simulink model "Test2_2"  (R2021a)
(part 2 of 3)

  Line 178 : spsDistributedParametersLineLib/Distributed Parameters Line  Phases=3  Length=0.02  Frequency=50  Resistance=[0.646656091154803 0.0486237908083191 0.0486712220507153;0.0486237908083191 0.646561225344642 0.0486237934466192;0.0486712220507153 0.0486237934466192 0.646656091154803]  Inductance=[0.00282448912315926 0.00133270803418135 0.00132951476746136;0.00133270803418135 0.00282479813276775 0.00133799988507366;0.00132951476746136 0.00133799988507366 0.00282448912315926]  Capacitance=[7.89543174552926e-09 -1.85986777702161e-09 -1.7901190036642e-09;-1.85986777702161e-09 7.82540023894543e-09 -1.8957321828871e-09;-1.7901190036642e-09 -1.8957321828871e-09 7.91264394645417e-09]  x1=[132.760320780997 9780.39904958768 9780.48623798031;314.159265358979 314.159265358979 314.159265358979;1.01437748390424 -0.192488813536579 -1.76345330045066]  x2=[132.762640557686 9780.24311209195 9780.33092876166;314.159265358979 314.159265358979 314.159265358979;1.01437617109871 -0.192497610718672 -1.7634621098678]  x3=[0.148387535223296 13.4653889012838 13.6374305581098;314.159265358979 314.159265358979 314.159265358979;0.608049237389297 -0.0518272275363164 -1.62927252881615]  x4=[0.112365930559543 36.4950552140708 36.6918967608298;314.159265358979 314.159265358979 314.159265358979;1.56346628767465 -0.244262443878478 -1.81321823531052]  x5=9.5829454252223e-08  V1=ones(3,3)  V2=ones(3,3)  I1=ones(3,3)  I2=ones(3,3)  nHarmo=1  Measurements=None  Decoupling=off  VsMag0=0  VrMag0=0  VsAngle0=0  VrAngle0=0  IsMag0=0  IrMag0=0  IsAngle0=0  IrAngle0=0
      settings: SourceProductBaseCode=PS
  Line 179 : spsDistributedParametersLineLib/Distributed Parameters Line  Phases=3  Length=1.15  Frequency=50  Resistance=[0.646656091154803 0.0486237908083191 0.0486712220507153;0.0486237908083191 0.646561225344642 0.0486237934466192;0.0486712220507153 0.0486237934466192 0.646656091154803]  Inductance=[0.00282448912315926 0.00133270803418135 0.00132951476746136;0.00133270803418135 0.00282479813276775 0.00133799988507366;0.00132951476746136 0.00133799988507366 0.00282448912315926]  Capacitance=[7.89543174552926e-09 -1.85986777702161e-09 -1.7901190036642e-09;-1.85986777702161e-09 7.82540023894543e-09 -1.8957321828871e-09;-1.7901190036642e-09 -1.8957321828871e-09 7.91264394645417e-09]  x1=[132.760320780997 9780.39904958768 9780.4862379803;314.159265358979 314.159265358979 314.159265358979;1.0126765112357 -0.193840124605235 -1.76480589787176]  x2=[132.768895455589 9779.25512812822 9779.34440600344;314.159265358979 314.159265358979 314.159265358979;1.01270315248622 -0.193874930127169 -1.76484031870729]  x3=[0.119132447239703 23.5945130394912 23.7849338463872;314.159265358979 314.159265358979 314.159265358979;0.986640133034939 -0.173292086707206 -1.74446117743403]  x4=[0.112976783804386 26.1275376195522 26.3187826598894;314.159265358979 314.159265358979 314.159265358979;1.03838062207725 -0.213738048990041 -1.78453527997739]  x5=5.51019361950282e-06  V1=ones(3,3)  V2=ones(3,3)  I1=ones(3,3)  I2=ones(3,3)  nHarmo=1  Measurements=None  Decoupling=off  VsMag0=0  VrMag0=0  VsAngle0=0  VrAngle0=0  IsMag0=0  IrMag0=0  IsAngle0=0  IrAngle0=0
      settings: SourceProductBaseCode=PS
  Line 18 : spsDistributedParametersLineLib/Distributed Parameters Line  Phases=3  Length=0.23002  Frequency=50  Resistance=[0.476003738225748 0.351747138225748 0.351747138225748;0.351747138225748 0.476003738225748 0.351747138225748;0.351747138225748 0.351747138225748 0.476003738225748]  Inductance=[0.000705954362986426 0.000459934243504405 0.000459934243504405;0.000459934243504405 0.000705954362986426 0.000459934243504405;0.000459934243504405 0.000459934243504405 0.000705954362986426]  Capacitance=[5.7561313269996e-07 -1.37543883484145e-07 -1.37543912800485e-07;-1.37543883484145e-07 5.75613027339387e-07 -1.37543875208088e-07;-1.37543912800485e-07 -1.37543875208088e-07 5.75613005057695e-07]  x1=[3.71917240590445 9847.49146197163 9847.74083952394;314.159265358979 314.159265358979 314.159265358979;1.3084049652874 2.1767138521056 -2.53557965242628]  x2=[3.71917715052359 9847.49597307011 9847.74535073597;314.159265358979 314.159265358979 314.159265358979;1.30840201930712 2.1767131156343 -2.53558038889746]  x3=[0.0504254137239255 529.580365853532 529.593736036669;314.159265358979 314.159265358979 314.159265358979;1.30680616940855 2.17575630443441 -2.53653720002242]  x4=[0.0504254137677653 529.58036594773 529.593736129492;314.159265358979 314.159265358979 314.159265358979;1.30840201941079 2.17671311563465 -2.53558038889797]  x5=5.08443513939426e-06  V1=ones(3,3)  V2=ones(3,3)  I1=ones(3,3)  I2=ones(3,3)  nHarmo=1  Measurements=None  Decoupling=off  VsMag0=0  VrMag0=0  VsAngle0=0  VrAngle0=0  IsMag0=0  IrMag0=0  IsAngle0=0  IrAngle0=0
      settings: SourceProductBaseCode=PS
  Line 180 : spsDistributedParametersLineLib/Distributed Parameters Line  Phases=3  Length=0.19  Frequency=50  Resistance=[0.646656091154803 0.0486237908083191 0.0486712220507153;0.0486237908083191 0.646561225344642 0.0486237934466192;0.0486712220507153 0.0486237934466192 0.646656091154803]  Inductance=[0.00282448912315926 0.00133270803418135 0.00132951476746136;0.00133270803418135 0.00282479813276775 0.00133799988507366;0.00132951476746136 0.00133799988507366 0.00282448912315926]  Capacitance=[7.89543174552926e-09 -1.85986777702161e-09 -1.7901190036642e-09;-1.85986777702161e-09 7.82540023894543e-09 -1.8957321828871e-09;-1.7901190036642e-09 -1.8957321828871e-09 7.91264394645417e-09]  x1=[132.768895455589 9779.25512812822 9779.34440600344;314.159265358979 314.159265358979 314.159265358979;1.01414822661171 -0.192726913644063 -1.76369120939378]  x2=[132.769311497012 9779.19565973239 9779.28506308661;314.159265358979 314.159265358979 314.159265358979;1.01414926755144 -0.192727707419426 -1.76369198402374]  x3=[0.116896171265332 24.525871144399 24.717022211576;314.159265358979 314.159265358979 314.159265358979;1.00614674760907 -0.184195073380317 -1.75522965039059]  x4=[0.115258964799221 25.2392564131172 25.4306773509319;314.159265358979 314.159265358979 314.159265358979;1.0219763695912 -0.201242395673975 -1.77214032483868]  x5=9.10379815396118e-07  V1=ones(3,3)  V2=ones(3,3)  I1=ones(3,3)  I2=ones(3,3)  nHarmo=1  Measurements=None  Decoupling=off  VsMag0=0  VrMag0=0  VsAngle0=0  VrAngle0=0  IsMag0=0  IrMag0=0  IsAngle0=0  IrAngle0=0
      settings: SourceProductBaseCode=PS
  Line 181 : spsDistributedParametersLineLib/Distributed Parameters Line  Phases=3  Length=0.34002  Frequency=50  Resistance=[0.646656091154803 0.0486237908083191 0.0486712220507153;0.0486237908083191 0.646561225344642 0.0486237934466192;0.0486712220507153 0.0486237934466192 0.646656091154803]  Inductance=[0.00282448912315926 0.00133270803418135 0.00132951476746136;0.00133270803418135 0.00282479813276775 0.00133799988507366;0.00132951476746136 0.00133799988507366 0.00282448912315926]  Capacitance=[7.89543174552926e-09 -1.85986777702161e-09 -1.7901190036642e-09;-1.85986777702161e-09 7.82540023894543e-09 -1.8957321828871e-09;-1.7901190036642e-09 -1.8957321828871e-09 7.91264394645417e-09]  x1=[132.768895455589 9779.25512812822 9779.34440600344;314.159265358979 314.159265358979 314.159265358979;1.01392240367389 -0.192906315136558 -1.76387078166379]  x2=[132.770600279391 9779.01933633328 9779.10899976005;314.159265358979 314.159265358979 314.159265358979;1.01392869633865 -0.192914667267989 -1.76387904990223]  x3=[0.118343745882774 23.9675286419785 24.1584478761822;314.159265358979 314.159265358979 314.159265358979;0.997308043857375 -0.179970297450305 -1.75105844200714]  x4=[0.113820605326666 25.7908196746096 25.9823125069988;314.159265358979 314.159265358979 314.159265358979;1.03068145843498 -0.205328116348918 -1.77618443924685]  x5=1.62919655174204e-06  V1=ones(3,3)  V2=ones(3,3)  I1=ones(3,3)  I2=ones(3,3)  nHarmo=1  Measurements=None  Decoupling=off  VsMag0=0  VrMag0=0  VsAngle0=0  VrAngle0=0  IsMag0=0  IrMag0=0  IsAngle0=0  IrAngle0=0
      settings: SourceProductBaseCode=PS
  Line 182 : spsDistributedParametersLineLib/Distributed Parameters Line  Phases=3  Length=0.12001  Frequency=50  Resistance=[0.646656091154803 0.0486237908083191 0.0486712220507153;0.0486237908083191 0.646561225344642 0.0486237934466192;0.0486712220507153 0.0486237934466192 0.646656091154803]  Inductance=[0.00282448912315926 0.00133270803418135 0.00132951476746136;0.00133270803418135 0.00282479813276775 0.00133799988507366;0.00132951476746136 0.00133799988507366 0.00282448912315926]  Capacitance=[7.89543174552926e-09 -1.85986777702161e-09 -1.7901190036642e-09;-1.85986777702161e-09 7.82540023894543e-09 -1.8957321828871e-09;-1.7901190036642e-09 -1.8957321828871e-09 7.91264394645417e-09]  x1=[132.770600279391 9779.01933633329 9779.10899976005;314.159265358979 314.159265358979 314.159265358979;1.01425987421193 -0.192651568198772 -1.76361570038133]  x2=[132.770823188964 9778.98793079047 9779.07766838742;314.159265358979 314.159265358979 314.159265358979;1.01426027694864 -0.192651696827363 -1.76361581957704]  x3=[0.116692617125028 24.6048761697535 24.7960740880757;314.159265358979 314.159265358979 314.159265358979;1.0071810631724 -0.184522294117927 -1.75555186557876]  x4=[0.115471698714884 25.1629262769793 25.3543559824755;314.159265358979 314.159265358979 314.159265358979;1.02123232994647 -0.200742607895418 -1.77164416592318]  x5=5.75024640240464e-07  V1=ones(3,3)  V2=ones(3,3)  I1=ones(3,3)  I2=ones(3,3)  nHarmo=1  Measurements=None  Decoupling=off  VsMag0=0  VrMag0=0  VsAngle0=0  VrAngle0=0  IsMag0=0  IrMag0=0  IsAngle0=0  IrAngle0=0
      settings: SourceProductBaseCode=PS
  Line 183 : spsDistributedParametersLineLib/Distributed Parameters Line  Phases=3  Length=0.82  Frequency=50  Resistance=[0.646656091154803 0.0486237908083191 0.0486712220507153;0.0486237908083191 0.646561225344642 0.0486237934466192;0.0486712220507153 0.0486237934466192 0.646656091154803]  Inductance=[0.00282448912315926 0.00133270803418135 0.00132951476746136;0.00133270803418135 0.00282479813276775 0.00133799988507366;0.00132951476746136 0.00133799988507366 0.00282448912315926]  Capacitance=[7.89543174552926e-09 -1.85986777702161e-09 -1.7901190036642e-09;-1.85986777702161e-09 7.82540023894543e-09 -1.8957321828871e-09;-1.7901190036642e-09 -1.8957321828871e-09 7.91264394645417e-09]  x1=[132.770600279391 9779.01933633329 9779.10899976005;314.159265358979 314.159265358979 314.159265358979;1.01320618938162 -0.193488651592532 -1.7644535806192]  x2=[132.773030713821 9778.65794538422 9778.74801773919;314.159265358979 314.159265358979 314.159265358979;1.01321912550127 -0.193506961178328 -1.76447174424821]  x3=[0.117696020207344 24.2308419112294 24.4216856976167;314.159265358979 314.159265358979 314.159265358979;1.00402501162747 -0.188531443558717 -1.7595499365372]  x4=[0.114394203828366 25.4954608594138 25.6866387013508;314.159265358979 314.159265358979 314.159265358979;1.02141318288896 -0.199174402225701 -1.77009111934403]  x5=3.92900762434114e-06  V1=ones(3,3)  V2=ones(3,3)  I1=ones(3,3)  I2=ones(3,3)  nHarmo=1  Measurements=None  Decoupling=off  VsMag0=0  VrMag0=0  VsAngle0=0  VrAngle0=0  IsMag0=0  IrMag0=0  IsAngle0=0  IrAngle0=0
      settings: SourceProductBaseCode=PS
  Line 184 : spsDistributedParametersLineLib/Distributed Parameters Line  Phases=3  Length=1.11  Frequency=50  Resistance=[0.646656091154803 0.0486237908083191 0.0486712220507153;0.0486237908083191 0.646561225344642 0.0486237934466192;0.0486712220507153 0.0486237934466192 0.646656091154803]  Inductance=[0.00282448912315926 0.00133270803418135 0.00132951476746136;0.00133270803418135 0.00282479813276775 0.00133799988507366;0.00132951476746136 0.00133799988507366 0.00282448912315926]  Capacitance=[7.89543174552926e-09 -1.85986777702161e-09 -1.7901190036642e-09;-1.85986777702161e-09 7.82540023894543e-09 -1.8957321828871e-09;-1.7901190036642e-09 -1.8957321828871e-09 7.91264394645417e-09]  x1=[132.622916358188 9790.14137890304 9790.19164885507;314.159265358979 314.159265358979 314.159265358979;1.01278515473274 -0.193268682744106 -1.76423408152936]  x2=[132.760320780997 9780.39904958768 9780.48623798031;314.159265358979 314.159265358979 314.159265358979;1.01273672265759 -0.193792290585105 -1.76475801831703]  x3=[0.152346754331472 12.2947814918702 12.4612185017915;314.159265358979 314.159265358979 314.159265358979;0.594199315329576 -0.00138291762119667 -1.58021705380452]  x4=[0.111382020462222 37.7484827942738 37.9443108810034;314.159265358979 314.159265358979 314.159265358979;1.60015314636976 -0.256645729486216 -1.82558858391367]  x5=5.31853471099837e-06  V1=ones(3,3)  V2=ones(3,3)  I1=ones(3,3)  I2=ones(3,3)  nHarmo=1  Measurements=None  Decoupling=off  VsMag0=0  VrMag0=0  VsAngle0=0  VrAngle0=0  IsMag0=0  IrMag0=0  IsAngle0=0  IrAngle0=0
      settings: SourceProductBaseCode=PS
  Line 185 : spsDistributedParametersLineLib/Distributed Parameters Line  Phases=3  Length=0.26  Frequency=50  Resistance=[0.646656091154803 0.0486237908083191 0.0486712220507153;0.0486237908083191 0.646561225344642 0.0486237934466192;0.0486712220507153 0.0486237934466192 0.646656091154803]  Inductance=[0.00282448912315926 0.00133270803418135 0.00132951476746136;0.00133270803418135 0.00282479813276775 0.00133799988507366;0.00132951476746136 0.00133799988507366 0.00282448912315926]  Capacitance=[7.89543174552926e-09 -1.85986777702161e-09 -1.7901190036642e-09;-1.85986777702161e-09 7.82540023894543e-09 -1.8957321828871e-09;-1.7901190036642e-09 -1.8957321828871e-09 7.91264394645417e-09]  x1=[132.813625527751 9776.5341567036 9775.93354168532;314.159265358979 314.159265358979 314.159265358979;1.06940231990873 2.2562343630252 -2.45590055419348]  x2=[132.813635699535 9776.5346292619 9775.93401511466;314.159265358979 314.159265358979 314.159265358979;1.06940228688053 2.25623430152678 -2.45590061621223]  x3=[0.116108906627122 24.8728268734641 25.0622687838346;314.159265358979 314.159265358979 314.159265358979;1.06901092913211 2.25592341114659 -2.45621180230919]  x4=[0.116108906656619 24.8728268736832 25.0622687839728;314.159265358979 314.159265358979 314.159265358979;1.06940228690124 2.25623430152497 -2.45590061621189]  x5=1.2457829052789e-06  V1=ones(3,3)  V2=ones(3,3)  I1=ones(3,3)  I2=ones(3,3)  nHarmo=1  Measurements=None  Decoupling=off  VsMag0=0  VrMag0=0  VsAngle0=0  VrAngle0=0  IsMag0=0  IrMag0=0  IsAngle0=0  IrAngle0=0
      settings: SourceProductBaseCode=PS
  Line 186 : spsDistributedParametersLineLib/Distributed Parameters Line  Phases=3  Length=0.20999  Frequency=50  Resistance=[0.646656091154803 0.0486237908083191 0.0486712220507153;0.0486237908083191 0.646561225344642 0.0486237934466192;0.0486712220507153 0.0486237934466192 0.646656091154803]  Inductance=[0.00282448912315926 0.00133270803418135 0.00132951476746136;0.00133270803418135 0.00282479813276775 0.00133799988507366;0.00132951476746136 0.00133799988507366 0.00282448912315926]  Capacitance=[7.89543174552926e-09 -1.85986777702161e-09 -1.7901190036642e-09;-1.85986777702161e-09 7.82540023894543e-09 -1.8957321828871e-09;-1.7901190036642e-09 -1.8957321828871e-09 7.91264394645417e-09]  x1=[132.622916358188 9790.14137890304 9790.19164885507;314.159265358979 314.159265358979 314.159265358979;1.01413992677824 -0.192192405332689 -1.76315677957806]  x2=[132.636539480394 9788.9974167178 9789.04732836895;314.159265358979 314.159265358979 314.159265358979;1.01420067383058 -0.19224254383873 -1.76320664889138]  x3=[0.150314506330029 17.4936829684655 17.6654938727302;314.159265358979 314.159265358979 314.159265358979;0.855909012601554 -0.0772116560117839 -1.64953774624993]  x4=[0.0867526882375548 32.4991450226245 32.7078437102462;314.159265358979 314.159265358979 314.159265358979;1.29031677246604 -0.254218771458032 -1.82466035998793]  x5=1.00616135492121e-06  V1=ones(3,3)  V2=ones(3,3)  I1=ones(3,3)  I2=ones(3,3)  nHarmo=1  Measurements=None  Decoupling=off  VsMag0=0  VrMag0=0  VsAngle0=0  VrAngle0=0  IsMag0=0  IrMag0=0  IsAngle0=0  IrAngle0=0
      settings: SourceProductBaseCode=PS
  Line 187 : spsDistributedParametersLineLib/Distributed Parameters Line  Phases=3  Length=0.23002  Frequency=50  Resistance=[0.476003738225748 0.351747138225748 0.351747138225748;0.351747138225748 0.476003738225748 0.351747138225748;0.351747138225748 0.351747138225748 0.476003738225748]  Inductance=[0.000705954362986426 0.000459934243504405 0.000459934243504405;0.000459934243504405 0.000705954362986426 0.000459934243504405;0.000459934243504405 0.000459934243504405 0.000705954362986426]  Capacitance=[5.7561313269996e-07 -1.37543883484145e-07 -1.37543912800485e-07;-1.37543883484145e-07 5.75613027339387e-07 -1.37543875208088e-07;-1.37543912800485e-07 -1.37543875208088e-07 5.75613005057695e-07]  x1=[5.39076266164301 9790.03085420358 9790.92794571974;314.159265358979 314.159265358979 314.159265358979;1.25651063342885 -0.11129659928421 -1.68211619564289]  x2=[5.39512619108942 9789.77536998703 9790.67197892186;314.159265358979 314.159265358979 314.159265358979;1.25599895948112 -0.111303669531063 -1.68212329506927]  x3=[0.0841543499142566 518.968404100205 518.999864130553;314.159265358979 314.159265358979 314.159265358979;1.0837782557924 -0.107425354639001 -1.67824483434028]  x4=[0.0649317655065428 534.007668121263 534.072589606561;314.159265358979 314.159265358979 314.159265358979;1.47871484672243 -0.116009851834134 -1.68682933238994]  x5=5.08443513939426e-06  V1=ones(3,3)  V2=ones(3,3)  I1=ones(3,3)  I2=ones(3,3)  nHarmo=1  Measurements=None  Decoupling=off  VsMag0=0  VrMag0=0  VsAngle0=0  VrAngle0=0  IsMag0=0  IrMag0=0  IsAngle0=0  IrAngle0=0
      settings: SourceProductBaseCode=PS
  Line 188 : spsDistributedParametersLineLib/Distributed Parameters Line  Phases=3  Length=0.02  Frequency=50  Resistance=[0.476003738225748 0.351747138225748 0.351747138225748;0.351747138225748 0.476003738225748 0.351747138225748;0.351747138225748 0.351747138225748 0.476003738225748]  Inductance=[0.000705954362986426 0.000459934243504405 0.000459934243504405;0.000459934243504405 0.000705954362986426 0.000459934243504405;0.000459934243504405 0.000459934243504405 0.000705954362986426]  Capacitance=[5.7561313269996e-07 -1.37543883484145e-07 -1.37543912800485e-07;-1.37543883484145e-07 5.75613027339387e-07 -1.37543875208088e-07;-1.37543912800485e-07 -1.37543875208088e-07 5.75613005057695e-07]  x1=[5.702815092939 9777.61936014807 9777.74195325645;314.159265358979 314.159265358979 314.159265358979;1.28271106732455 2.1748176079715 -2.53747364786867]  x2=[5.70282059813833 9777.61614892348 9777.73874302418;314.159265358979 314.159265358979 314.159265358979;1.28270811564057 2.17481740369348 -2.53747385225643]  x3=[0.0774549361110471 525.08480858354 525.091457447942;314.159265358979 314.159265358979 314.159265358979;1.2737863091309 2.17477593478717 -2.53751626872189]  x4=[0.0775822635703045 527.668783896918 527.675253276444;314.159265358979 314.159265358979 314.159265358979;1.29147944151647 2.17477584854756 -2.53751446436691]  x5=4.42086352438419e-07  V1=ones(3,3)  V2=ones(3,3)  I1=ones(3,3)  I2=ones(3,3)  nHarmo=1  Measurements=None  Decoupling=off  VsMag0=0  VrMag0=0  VsAngle0=0  VrAngle0=0  IsMag0=0  IrMag0=0  IsAngle0=0  IrAngle0=0
      settings: SourceProductBaseCode=PS
  Line 189 : spsDistributedParametersLineLib/Distributed Parameters Line  Phases=3  Length=0.23  Frequency=50  Resistance=[0.646656091154803 0.0486237908083191 0.0486712220507153;0.0486237908083191 0.646561225344642 0.0486237934466192;0.0486712220507153 0.0486237934466192 0.646656091154803]  Inductance=[0.00282448912315926 0.00133270803418135 0.00132951476746136;0.00133270803418135 0.00282479813276775 0.00133799988507366;0.00132951476746136 0.00133799988507366 0.00282448912315926]  Capacitance=[7.89543174552926e-09 -1.85986777702161e-09 -1.7901190036642e-09;-1.85986777702161e-09 7.82540023894543e-09 -1.8957321828871e-09;-1.7901190036642e-09 -1.8957321828871e-09 7.91264394645417e-09]  x1=[133.135076792434 9757.65693831808 9757.85248417411;314.159265358979 314.159265358979 314.159265358979;1.01347027244292 -0.194011574894598 -1.76498104996715]  x2=[133.155335063346 9756.76318303855 9756.96500336632;314.159265358979 314.159265358979 314.159265358979;1.01342220404239 -0.194062538224466 -1.76503251692427]  x3=[0.130895185238685 19.0742229411415 19.2550712168771;314.159265358979 314.159265358979 314.159265358979;0.629519876058864 -0.145810884155953 -1.72036784457314]  x4=[0.121727423189322 30.6109982798558 30.8075650917927;314.159265358979 314.159265358979 314.159265358979;1.42762978343165 -0.224303632259894 -1.79312462393561]  x5=1.10203872390056e-06  V1=ones(3,3)  V2=ones(3,3)  I1=ones(3,3)  I2=ones(3,3)  nHarmo=1  Measurements=None  Decoupling=off  VsMag0=0  VrMag0=0  VsAngle0=0  VrAngle0=0  IsMag0=0  IrMag0=0  IsAngle0=0  IrAngle0=0
      settings: SourceProductBaseCode=PS
  Line 19 : spsDistributedParametersLineLib/Distributed Parameters Line  Phases=3  Length=0.24001  Frequency=50  Resistance=[0.646656091154803 0.0486237908083191 0.0486712220507153;0.0486237908083191 0.646561225344642 0.0486237934466192;0.0486712220507153 0.0486237934466192 0.646656091154803]  Inductance=[0.00282448912315926 0.00133270803418135 0.00132951476746136;0.00133270803418135 0.00282479813276775 0.00133799988507366;0.00132951476746136 0.00133799988507366 0.00282448912315926]  Capacitance=[7.89543174552926e-09 -1.85986777702161e-09 -1.7901190036642e-09;-1.85986777702161e-09 7.82540023894543e-09 -1.8957321828871e-09;-1.7901190036642e-09 -1.8957321828871e-09 7.91264394645417e-09]  x1=[131.672741119116 9858.70653543795 9858.14819692635;314.159265358979 314.159265358979 314.159265358979;1.0693438076424 2.25972015370559 -2.45242843951262]  x2=[131.708950173583 9855.73083509479 9855.1889775783;314.159265358979 314.159265358979 314.159265358979;1.06940916271926 2.25953652137496 -2.45260951181303]  x3=[0.177403325432903 6.54675155696578 6.81994292571319;314.159265358979 314.159265358979 314.159265358979;0.686154791444632 2.61467560589239 -2.11231114596141]  x4=[0.0933481039457772 44.0780759081465 44.1696303796175;314.159265358979 314.159265358979 314.159265358979;1.8590907667426 2.20780897138387 -2.50422818268227]  x5=1.1500013657538e-06  V1=ones(3,3)  V2=ones(3,3)  I1=ones(3,3)  I2=ones(3,3)  nHarmo=1  Measurements=None  Decoupling=off  VsMag0=0  VrMag0=0  VsAngle0=0  VrAngle0=0  IsMag0=0  IrMag0=0  IsAngle0=0  IrAngle0=0
      settings: SourceProductBaseCode=PS
  Line 190 : spsDistributedParametersLineLib/Distributed Parameters Line  Phases=3  Length=1.62  Frequency=50  Resistance=[0.80718830189013 0.0486237908083191 0.0486712220507153;0.0486237908083191 0.807093436079969 0.0486237934466192;0.0486712220507153 0.0486237934466192 0.80718830189013]  Inductance=[0.00279786707424938 0.00133270803418135 0.00132951476746136;0.00133270803418135 0.00279817608385787 0.00133799988507366;0.00132951476746136 0.00133799988507366 0.00279786707424938]  Capacitance=[7.73340098830622e-09 -1.79942827973291e-09 -1.73218055098733e-09;-1.79942827973291e-09 7.66505189233746e-09 -1.83375898618858e-09;-1.73218055098733e-09 -1.83375898618858e-09 7.749673531177e-09]  x1=[57.0469952701758 9757.74181875468 9758.02095017472;314.159265358979 314.159265358979 314.159265358979;1.07791383820645 -0.199946323437713 -1.77087760749933]  x2=[57.0474438101102 9757.7357305126 9758.01492341474;314.159265358979 314.159265358979 314.159265358979;1.07791469091692 -0.199949631400151 -1.77088093293837]  x3=[0.0497475444738988 24.6964027146535 24.885037948888;314.159265358979 314.159265358979 314.159265358979;1.07431084552759 -0.201582781638177 -1.77251775708706]  x4=[0.0495871378111349 24.7268757699296 24.9155196269109;314.159265358979 314.159265358979 314.159265358979;1.07910423737049 -0.200213547154174 -1.77114277061765]  x5=7.70442045759223e-06  V1=ones(3,3)  V2=ones(3,3)  I1=ones(3,3)  I2=ones(3,3)  nHarmo=1  Measurements=None  Decoupling=off  VsMag0=0  VrMag0=0  VsAngle0=0  VrAngle0=0  IsMag0=0  IrMag0=0  IsAngle0=0  IrAngle0=0
      settings: SourceProductBaseCode=PS
  Line 191 : spsDistributedParametersLineLib/Distributed Parameters Line  Phases=3  Length=0.54002  Frequency=50  Resistance=[0.646656091154803 0.0486237908083191 0.0486712220507153;0.0486237908083191 0.646561225344642 0.0486237934466192;0.0486712220507153 0.0486237934466192 0.646656091154803]  Inductance=[0.00282448912315926 0.00133270803418135 0.00132951476746136;0.00133270803418135 0.00282479813276775 0.00133799988507366;0.00132951476746136 0.00133799988507366 0.00282448912315926]  Capacitance=[7.89543174552926e-09 -1.85986777702161e-09 -1.7901190036642e-09;-1.85986777702161e-09 7.82540023894543e-09 -1.8957321828871e-09;-1.7901190036642e-09 -1.8957321828871e-09 7.91264394645417e-09]  x1=[133.087156904702 9759.74726224708 9759.92804024952;314.159265358979 314.159265358979 314.159265358979;1.01311734999931 -0.194260576934043 -1.76522920894174]  x2=[133.135076792434 9757.65693831808 9757.85248417411;314.159265358979 314.159265358979 314.159265358979;1.01300360381753 -0.194382312467611 -1.76535214045608]  x3=[0.131017257846132 19.0543485504157 19.2352442248447;314.159265358979 314.159265358979 314.159265358979;0.626338806959044 -0.148951964517859 -1.72351123138487]  x4=[0.121796683859199 30.6169679505761 30.8134856249678;314.159265358979 314.159265358979 314.159265358979;1.4299626434303 -0.223074835577922 -1.79189170469167]  x5=2.58749109426427e-06  V1=ones(3,3)  V2=ones(3,3)  I1=ones(3,3)  I2=ones(3,3)  nHarmo=1  Measurements=None  Decoupling=off  VsMag0=0  VrMag0=0  VsAngle0=0  VrAngle0=0  IsMag0=0  IrMag0=0  IsAngle0=0  IrAngle0=0
      settings: SourceProductBaseCode=PS
  Line 192 : spsDistributedParametersLineLib/Distributed Parameters Line  Phases=3  Length=0.13998  Frequency=50  Resistance=[0.646656091154803 0.0486237908083191 0.0486712220507153;0.0486237908083191 0.646561225344642 0.0486237934466192;0.0486712220507153 0.0486237934466192 0.646656091154803]  Inductance=[0.00282448912315926 0.00133270803418135 0.00132951476746136;0.00133270803418135 0.00282479813276775 0.00133799988507366;0.00132951476746136 0.00133799988507366 0.00282448912315926]  Capacitance=[7.89543174552926e-09 -1.85986777702161e-09 -1.7901190036642e-09;-1.85986777702161e-09 7.82540023894543e-09 -1.8957321828871e-09;-1.7901190036642e-09 -1.8957321828871e-09 7.91264394645417e-09]  x1=[133.087156904702 9759.74726224708 9759.92804024952;314.159265358979 314.159265358979 314.159265358979;1.01371952442968 -0.193782188898729 -1.7647503655149]  x2=[133.088589823031 9759.52716144075 9759.70818846233;314.159265358979 314.159265358979 314.159265358979;1.01372725084576 -0.193792510709673 -1.76476059726163]  x3=[0.122163810645742 22.6294782968273 22.8199514892167;314.159265358979 314.159265358979 314.159265358979;0.985278409185769 -0.170289808578383 -1.7414782208149]  x4=[0.110650305907688 27.0485535390112 27.2403024111394;314.159265358979 314.159265358979 314.159265358979;1.04490739366276 -0.213599145126494 -1.78440892060145]  x5=6.70710350311308e-07  V1=ones(3,3)  V2=ones(3,3)  I1=ones(3,3)  I2=ones(3,3)  nHarmo=1  Measurements=None  Decoupling=off  VsMag0=0  VrMag0=0  VsAngle0=0  VrAngle0=0  IsMag0=0  IrMag0=0  IsAngle0=0  IrAngle0=0
      settings: SourceProductBaseCode=PS
  Line 193 : spsDistributedParametersLineLib/Distributed Parameters Line  Phases=3  Length=0.14997  Frequency=50  Resistance=[0.476003738225748 0.351747138225748 0.351747138225748;0.351747138225748 0.476003738225748 0.351747138225748;0.351747138225748 0.351747138225748 0.476003738225748]  Inductance=[0.000705954362986426 0.000459934243504405 0.000459934243504405;0.000459934243504405 0.000705954362986426 0.000459934243504405;0.000459934243504405 0.000459934243504405 0.000705954362986426]  Capacitance=[5.7561313269996e-07 -1.37543883484145e-07 -1.37543912800485e-07;-1.37543883484145e-07 5.75613027339387e-07 -1.37543875208088e-07;-1.37543912800485e-07 -1.37543875208088e-07 5.75613005057695e-07]  x1=[6.23421972802901 9760.56111335783 9761.57727591969;314.159265358979 314.159265358979 314.159265358979;1.24438681831645 -0.112596276927518 -1.68342184913864]  x2=[6.23422310991035 9760.5118175976 9761.52797502703;314.159265358979 314.159265358979 314.159265358979;1.2443855678239 -0.112597566638265 -1.68342313884934]  x3=[0.0846063798147464 522.907040647717 522.961439425086;314.159265358979 314.159265358979 314.159265358979;1.24334536406638 -0.111572946637743 -1.68239851867086]  x4=[0.08460632297266 527.32332143546 527.378179987414;314.159265358979 314.159265358979 314.159265358979;1.24438496302749 -0.114233932189958 -1.6850595045286]  x5=3.31498451375949e-06  V1=ones(3,3)  V2=ones(3,3)  I1=ones(3,3)  I2=ones(3,3)  nHarmo=1  Measurements=None  Decoupling=off  VsMag0=0  VrMag0=0  VsAngle0=0  VrAngle0=0  IsMag0=0  IrMag0=0  IsAngle0=0  IrAngle0=0
      settings: SourceProductBaseCode=PS
  Line 194 : spsDistributedParametersLineLib/Distributed Parameters Line  Phases=3  Length=1.7101  Frequency=50  Resistance=[0.646656091154803 0.0486237908083191 0.0486712220507153;0.0486237908083191 0.646561225344642 0.0486237934466192;0.0486712220507153 0.0486237934466192 0.646656091154803]  Inductance=[0.00282448912315926 0.00133270803418135 0.00132951476746136;0.00133270803418135 0.00282479813276775 0.00133799988507366;0.00132951476746136 0.00133799988507366 0.00282448912315926]  Capacitance=[7.89543174552926e-09 -1.85986777702161e-09 -1.7901190036642e-09;-1.85986777702161e-09 7.82540023894543e-09 -1.8957321828871e-09;-1.7901190036642e-09 -1.8957321828871e-09 7.91264394645417e-09]  x1=[132.809449296114 9777.81056053905 9777.20984376857;314.159265358979 314.159265358979 314.159265358979;1.0671373390958 2.25461316766885 -2.45752404891205]  x2=[132.813456590574 9776.52747960268 9775.92685411162;314.159265358979 314.159265358979 314.159265358979;1.0672218160218 2.2545019974351 -2.45763456671143]  x3=[0.11972938488699 23.544486948557 23.7331752047722;314.159265358979 314.159265358979 314.159265358979;1.06787796596569 2.2515247145875 -2.46061205879326]  x4=[0.112321414059214 26.1222679379442 26.3112414289237;314.159265358979 314.159265358979 314.159265358979;1.06377531428613 2.25534578400232 -2.45679167137988]  x5=8.19389748583632e-06  V1=ones(3,3)  V2=ones(3,3)  I1=ones(3,3)  I2=ones(3,3)  nHarmo=1  Measurements=None  Decoupling=off  VsMag0=0  VrMag0=0  VsAngle0=0  VrAngle0=0  IsMag0=0  IrMag0=0  IsAngle0=0  IrAngle0=0
      settings: SourceProductBaseCode=PS
  Line 195 : spsDistributedParametersLineLib/Distributed Parameters Line  Phases=3  Length=0.50001  Frequency=50  Resistance=[0.646656091154803 0.0486237908083191 0.0486712220507153;0.0486237908083191 0.646561225344642 0.0486237934466192;0.0486712220507153 0.0486237934466192 0.646656091154803]  Inductance=[0.00282448912315926 0.00133270803418135 0.00132951476746136;0.00133270803418135 0.00282479813276775 0.00133799988507366;0.00132951476746136 0.00133799988507366 0.00282448912315926]  Capacitance=[7.89543174552926e-09 -1.85986777702161e-09 -1.7901190036642e-09;-1.85986777702161e-09 7.82540023894543e-09 -1.8957321828871e-09;-1.7901190036642e-09 -1.8957321828871e-09 7.91264394645417e-09]  x1=[133.037581249628 9762.46497797497 9762.63118730738;314.159265358979 314.159265358979 314.159265358979;1.01325565136519 -0.194062675167044 -1.76503047147715]  x2=[133.087156904702 9759.74726224708 9759.92804024952;314.159265358979 314.159265358979 314.159265358979;1.01317757647406 -0.194212730955408 -1.76518131741713]  x3=[0.137657551528371 16.8897328513076 17.0673751370128;314.159265358979 314.159265358979 314.159265358979;0.618165192204538 -0.112215430794762 -1.68765061643102]  x4=[0.118078890205565 32.8501757890289 33.0463884024766;314.159265358979 314.159265358979 314.159265358979;1.47766209631206 -0.236675273740321 -1.80553319920578]  x5=2.3957842710327e-06  V1=ones(3,3)  V2=ones(3,3)  I1=ones(3,3)  I2=ones(3,3)  nHarmo=1  Measurements=None  Decoupling=off  VsMag0=0  VrMag0=0  VsAngle0=0  VrAngle0=0  IsMag0=0  IrMag0=0  IsAngle0=0  IrAngle0=0
      settings: SourceProductBaseCode=PS
  Line 196 : spsDistributedParametersLineLib/Distributed Parameters Line  Phases=3  Length=0.17  Frequency=50  Resistance=[0.646656091154803 0.0486237908083191 0.0486712220507153;0.0486237908083191 0.646561225344642 0.0486237934466192;0.0486712220507153 0.0486237934466192 0.646656091154803]  Inductance=[0.00282448912315926 0.00133270803418135 0.00132951476746136;0.00133270803418135 0.00282479813276775 0.00133799988507366;0.00132951476746136 0.00133799988507366 0.00282448912315926]  Capacitance=[7.89543174552926e-09 -1.85986777702161e-09 -1.7901190036642e-09;-1.85986777702161e-09 7.82540023894543e-09 -1.8957321828871e-09;-1.7901190036642e-09 -1.8957321828871e-09 7.91264394645417e-09]  x1=[133.037581249628 9762.46497797497 9762.63118730739;314.159265358979 314.159265358979 314.159265358979;1.01375241064868 -0.193668032542471 -1.76463545318074]  x2=[133.038492843106 9762.32402753733 9762.49040755994;314.159265358979 314.159265358979 314.159265358979;1.01375717981103 -0.193674281282447 -1.76464164528153]  x3=[0.119284477597522 23.6927854890215 23.8836043746308;314.159265358979 314.159265358979 314.159265358979;0.998219708030887 -0.180997275496016 -1.7520787523616]  x4=[0.113364938933958 25.989717439309 26.1812047273945;314.159265358979 314.159265358979 314.159265358979;1.0298385546531 -0.205419209990531 -1.7762906482843]  x5=8.14550361143895e-07  V1=ones(3,3)  V2=ones(3,3)  I1=ones(3,3)  I2=ones(3,3)  nHarmo=1  Measurements=None  Decoupling=off  VsMag0=0  VrMag0=0  VsAngle0=0  VrAngle0=0  IsMag0=0  IrMag0=0  IsAngle0=0  IrAngle0=0
      settings: SourceProductBaseCode=PS
  Line 197 : spsDistributedParametersLineLib/Distributed Parameters Line  Phases=3  Length=0.27999  Frequency=50  Resistance=[0.646656091154803 0.0486237908083191 0.0486712220507153;0.0486237908083191 0.646561225344642 0.0486237934466192;0.0486712220507153 0.0486237934466192 0.646656091154803]  Inductance=[0.00282448912315926 0.00133270803418135 0.00132951476746136;0.00133270803418135 0.00282479813276775 0.00133799988507366;0.00132951476746136 0.00133799988507366 0.00282448912315926]  Capacitance=[7.89543174552926e-09 -1.85986777702161e-09 -1.7901190036642e-09;-1.85986777702161e-09 7.82540023894543e-09 -1.8957321828871e-09;-1.7901190036642e-09 -1.8957321828871e-09 7.91264394645417e-09]  x1=[133.008279258237 9764.21720820124 9764.37497580907;314.159265358979 314.159265358979 314.159265358979;1.01362286312373 -0.19370504443354 -1.7646722390336]  x2=[133.037581249628 9762.46497797497 9762.63118730738;314.159265358979 314.159265358979 314.159265358979;1.01358684429132 -0.193799564139322 -1.76476710998636]  x3=[0.141111418839714 15.7831046686625 15.958587158098;314.159265358979 314.159265358979 314.159265358979;0.614101116600165 -0.0874560448517488 -1.66349319029285]  x4=[0.116319642948493 34.0250069092961 34.2211713325166;314.159265358979 314.159265358979 314.159265358979;1.50452893213982 -0.243231548135761 -1.81210760328089]  x5=1.341564444804e-06  V1=ones(3,3)  V2=ones(3,3)  I1=ones(3,3)  I2=ones(3,3)  nHarmo=1  Measurements=None  Decoupling=off  VsMag0=0  VrMag0=0  VsAngle0=0  VrAngle0=0  IsMag0=0  IrMag0=0  IsAngle0=0  IrAngle0=0
      settings: SourceProductBaseCode=PS
  Line 198 : spsDistributedParametersLineLib/Distributed Parameters Line  Phases=3  Length=0.28003  Frequency=50  Resistance=[0.476003738225748 0.351747138225748 0.351747138225748;0.351747138225748 0.476003738225748 0.351747138225748;0.351747138225748 0.351747138225748 0.476003738225748]  Inductance=[0.000705954362986426 0.000459934243504405 0.000459934243504405;0.000459934243504405 0.000705954362986426 0.000459934243504405;0.000459934243504405 0.000459934243504405 0.000705954362986426]  Capacitance=[5.7561313269996e-07 -1.37543883484145e-07 -1.37543912800485e-07;-1.37543883484145e-07 5.75613027339387e-07 -1.37543875208088e-07;-1.37543912800485e-07 -1.37543875208088e-07 5.75613005057695e-07]  x1=[6.50811897326202 9752.0600676398 9753.11034638649;314.159265358979 314.159265358979 314.159265358979;1.24492082205445 -0.113840594625838 -1.68466856137944]  x2=[6.50813752864608 9752.06722463642 9753.11750709961;314.159265358979 314.159265358979 314.159265358979;1.24490461777175 -0.113841774324923 -1.68466974190294]  x3=[0.0881172791660225 524.316841316303 524.373226476001;314.159265358979 314.159265358979 314.159265358979;1.24067027256394 -0.115053539136208 -1.68588189577737]  x4=[0.0882549063505425 524.316798965635 524.37326915554;314.159265358979 314.159265358979 314.159265358979;1.24720328025548 -0.113794660967974 -1.68462223867023]  x5=6.18987206366653e-06  V1=ones(3,3)  V2=ones(3,3)  I1=ones(3,3)  I2=ones(3,3)  nHarmo=1  Measurements=None  Decoupling=off  VsMag0=0  VrMag0=0  VsAngle0=0  VrAngle0=0  IsMag0=0  IrMag0=0  IsAngle0=0  IrAngle0=0
      settings: SourceProductBaseCode=PS
  Line 199 : spsDistributedParametersLineLib/Distributed Parameters Line  Phases=3  Length=0.28002  Frequency=50  Resistance=[0.646656091154803 0.0486237908083191 0.0486712220507153;0.0486237908083191 0.646561225344642 0.0486237934466192;0.0486712220507153 0.0486237934466192 0.646656091154803]  Inductance=[0.00282448912315926 0.00133270803418135 0.00132951476746136;0.00133270803418135 0.00282479813276775 0.00133799988507366;0.00132951476746136 0.00133799988507366 0.00282448912315926]  Capacitance=[7.89543174552926e-09 -1.85986777702161e-09 -1.7901190036642e-09;-1.85986777702161e-09 7.82540023894543e-09 -1.8957321828871e-09;-1.7901190036642e-09 -1.8957321828871e-09 7.91264394645417e-09]  x1=[133.241705638299 9751.03254736617 9751.25235319998;314.159265358979 314.159265358979 314.159265358979;1.01339304722221 -0.194664514681177 -1.76563459647833]  x2=[133.24176346223 9751.03525408047 9751.25506497785;314.159265358979 314.159265358979 314.159265358979;1.01339286180741 -0.194664867860082 -1.7656349526102]  x3=[0.116482494851082 24.8073915020261 24.9984304170338;314.159265358979 314.159265358979 314.159265358979;1.01215416178574 -0.195661008101636 -1.76663197055893]  x4=[0.116481684824936 24.807391941253 24.9984300051287;314.159265358979 314.159265358979 314.159265358979;1.01421022523785 -0.194003272179205 -1.7649727953082]  x5=1.34170818898537e-06  V1=ones(3,3)  V2=ones(3,3)  I1=ones(3,3)  I2=ones(3,3)  nHarmo=1  Measurements=None  Decoupling=off  VsMag0=0  VrMag0=0  VsAngle0=0  VrAngle0=0  IsMag0=0  IrMag0=0  IsAngle0=0  IrAngle0=0
      settings: SourceProductBaseCode=PS
  Line 2 : spsDistributedParametersLineLib/Distributed Parameters Line  Phases=3  Length=0.24001  Frequency=50  Resistance=[0.646656091154803 0.0486237908083191 0.0486712220507153;0.0486237908083191 0.646561225344642 0.0486237934466192;0.0486712220507153 0.0486237934466192 0.646656091154803]  Inductance=[0.00282448912315926 0.00133270803418135 0.00132951476746136;0.00133270803418135 0.00282479813276775 0.00133799988507366;0.00132951476746136 0.00133799988507366 0.00282448912315926]  Capacitance=[7.89543174552926e-09 -1.85986777702161e-09 -1.7901190036642e-09;-1.85986777702161e-09 7.82540023894543e-09 -1.8957321828871e-09;-1.7901190036642e-09 -1.8957321828871e-09 7.91264394645417e-09]  x1=[131.763809776127 9846.88411593864 9846.39278960383;314.159265358979 314.159265358979 314.159265358979;1.0696134193504 2.259071906178 -2.45306833697313]  x2=[131.767945414111 9846.3421209356 9845.85604977773;314.159265358979 314.159265358979 314.159265358979;1.06962257767498 2.25903805015682 -2.45310170021886]  x3=[0.121519007127094 21.5930955697861 21.8127920503779;314.159265358979 314.159265358979 314.159265358979;1.00870168408395 2.27738449714046 -2.4352453765687]  x4=[0.109342231555222 28.516753754079 28.6790058456149;314.159265358979 314.159265358979 314.159265358979;1.1369465508721 2.24492387551914 -2.46690617446182]  x5=1.1500013657538e-06  V1=ones(3,3)  V2=ones(3,3)  I1=ones(3,3)  I2=ones(3,3)  nHarmo=1  Measurements=None  Decoupling=off  VsMag0=0  VrMag0=0  VsAngle0=0  VrAngle0=0  IsMag0=0  IrMag0=0  IsAngle0=0  IrAngle0=0
      settings: SourceProductBaseCode=PS
  Line 20 : spsDistributedParametersLineLib/Distributed Parameters Line  Phases=3  Length=0.02  Frequency=50  Resistance=[0.646656091154803 0.0486237908083191 0.0486712220507153;0.0486237908083191 0.646561225344642 0.0486237934466192;0.0486712220507153 0.0486237934466192 0.646656091154803]  Inductance=[0.00282448912315926 0.00133270803418135 0.00132951476746136;0.00133270803418135 0.00282479813276775 0.00133799988507366;0.00132951476746136 0.00133799988507366 0.00282448912315926]  Capacitance=[7.89543174552926e-09 -1.85986777702161e-09 -1.7901190036642e-09;-1.85986777702161e-09 7.82540023894543e-09 -1.8957321828871e-09;-1.7901190036642e-09 -1.8957321828871e-09 7.91264394645417e-09]  x1=[131.672741119116 9858.70653543795 9858.14819692635;314.159265358979 314.159265358979 314.159265358979;1.06967498551568 2.25998325277481 -2.45216508999172]  x2=[131.672763250035 9858.70111309796 9858.14278418561;314.159265358979 314.159265358979 314.159265358979;1.06967523902033 2.25998313265772 -2.45216520792254]  x3=[0.11617622276114 24.7608381927207 24.9520932703347;314.159265358979 314.159265358979 314.159265358979;1.06802947857145 2.26639654673525 -2.44579649420859]  x4=[0.114074028569093 25.4176636213966 25.6089218370655;314.159265358979 314.159265358979 314.159265358979;1.07132068964814 2.25371196212684 -2.45839408854188]  x5=9.5829454252223e-08  V1=ones(3,3)  V2=ones(3,3)  I1=ones(3,3)  I2=ones(3,3)  nHarmo=1  Measurements=None  Decoupling=off  VsMag0=0  VrMag0=0  VsAngle0=0  VrAngle0=0  IsMag0=0  IrMag0=0  IsAngle0=0  IrAngle0=0
      settings: SourceProductBaseCode=PS
  Line 200 : spsDistributedParametersLineLib/Distributed Parameters Line  Phases=3  Length=0.3  Frequency=50  Resistance=[0.80718830189013 0.0486237908083191 0.0486712220507153;0.0486237908083191 0.807093436079969 0.0486237934466192;0.0486712220507153 0.0486237934466192 0.80718830189013]  Inductance=[0.00279786707424938 0.00133270803418135 0.00132951476746136;0.00133270803418135 0.00279817608385787 0.00133799988507366;0.00132951476746136 0.00133799988507366 0.00279786707424938]  Capacitance=[7.73340098830622e-09 -1.79942827973291e-09 -1.73218055098733e-09;-1.79942827973291e-09 7.66505189233746e-09 -1.83375898618858e-09;-1.73218055098733e-09 -1.83375898618858e-09 7.749673531177e-09]  x1=[57.210029617587 9751.12004846424 9751.42404795869;314.159265358979 314.159265358979 314.159265358979;1.08043806892435 -0.198993225133981 -1.76992375887121]  x2=[57.2100353645018 9751.12065081881 9751.42465135036;314.159265358979 314.159265358979 314.159265358979;1.08043801600358 -0.198993326632521 -1.769923861215]  x3=[0.0498477409283975 24.7419642762415 24.9312543642923;314.159265358979 314.159265358979 314.159265358979;1.07998981724863 -0.199344766599222 -1.77027559772855]  x4=[0.0498477409204113 24.7419642765517 24.9312543645246;314.159265358979 314.159265358979 314.159265358979;1.0804380161156 -0.198993326633706 -1.76992386121489]  x5=1.42674452918375e-06  V1=ones(3,3)  V2=ones(3,3)  I1=ones(3,3)  I2=ones(3,3)  nHarmo=1  Measurements=None  Decoupling=off  VsMag0=0  VrMag0=0  VsAngle0=0  VrAngle0=0  IsMag0=0  IrMag0=0  IsAngle0=0  IrAngle0=0
      settings: SourceProductBaseCode=PS
  Line 201 : spsDistributedParametersLineLib/Distributed Parameters Line  Phases=3  Length=0.26  Frequency=50  Resistance=[0.646656091154803 0.0486237908083191 0.0486712220507153;0.0486237908083191 0.646561225344642 0.0486237934466192;0.0486712220507153 0.0486237934466192 0.646656091154803]  Inductance=[0.00282448912315926 0.00133270803418135 0.00132951476746136;0.00133270803418135 0.00282479813276775 0.00133799988507366;0.00132951476746136 0.00133799988507366 0.00282448912315926]  Capacitance=[7.89543174552926e-09 -1.85986777702161e-09 -1.7901190036642e-09;-1.85986777702161e-09 7.82540023894543e-09 -1.8957321828871e-09;-1.7901190036642e-09 -1.8957321828871e-09 7.91264394645417e-09]  x1=[133.24176346223 9751.03525408047 9751.25506497785;314.159265358979 314.159265358979 314.159265358979;1.01342299762407 -0.194640926933007 -1.76561098889306]  x2=[133.241773666799 9751.03572540628 9751.25553721207;314.159265358979 314.159265358979 314.159265358979;1.01342296459584 -0.194640988431425 -1.76561105091181]  x3=[0.116483195220923 24.807954212143 24.9990013103188;314.159265358979 314.159265358979 314.159265358979;1.01303160685863 -0.194951878813149 -1.76592223701211]  x4=[0.11648319527517 24.8079542121287 24.9990013104482;314.159265358979 314.159265358979 314.159265358979;1.01342296460163 -0.194640988432029 -1.76561105090782]  x5=1.2457829052789e-06  V1=ones(3,3)  V2=ones(3,3)  I1=ones(3,3)  I2=ones(3,3)  nHarmo=1  Measurements=None  Decoupling=off  VsMag0=0  VrMag0=0  VsAngle0=0  VrAngle0=0  IsMag0=0  IrMag0=0  IsAngle0=0  IrAngle0=0
      settings: SourceProductBaseCode=PS
  Line 202 : spsDistributedParametersLineLib/Distributed Parameters Line  Phases=3  Length=0.02  Frequency=50  Resistance=[0.476003738225748 0.351747138225748 0.351747138225748;0.351747138225748 0.476003738225748 0.351747138225748;0.351747138225748 0.351747138225748 0.476003738225748]  Inductance=[0.000705954362986426 0.000459934243504405 0.000459934243504405;0.000459934243504405 0.000705954362986426 0.000459934243504405;0.000459934243504405 0.000459934243504405 0.000705954362986426]  Capacitance=[5.7561313269996e-07 -1.37543883484145e-07 -1.37543912800485e-07;-1.37543883484145e-07 5.75613027339387e-07 -1.37543875208088e-07;-1.37543912800485e-07 -1.37543875208088e-07 5.75613005057695e-07]  x1=[6.50811591516597 9752.06318197098 9753.11346054809;314.159265358979 314.159265358979 314.159265358979;1.24672929269148 -0.112758139533049 -1.68358610622703]  x2=[6.50811897326202 9752.0600676398 9753.11034638649;314.159265358979 314.159265358979 314.159265358979;1.24672654219093 -0.112758534941927 -1.68358650177918]  x3=[0.0882967777896706 523.402007382998 523.458231092664;314.159265358979 314.159265358979 314.159265358979;1.23888858861266 -0.113863509531861 -1.68469242505499]  x4=[0.0886317494304943 526.600553423609 526.657332891823;314.159265358979 314.159265358979 314.159265358979;1.25439898616315 -0.111742853488464 -1.68256987767727]  x5=4.42086352438419e-07  V1=ones(3,3)  V2=ones(3,3)  I1=ones(3,3)  I2=ones(3,3)  nHarmo=1  Measurements=None  Decoupling=off  VsMag0=0  VrMag0=0  VsAngle0=0  VrAngle0=0  IsMag0=0  IrMag0=0  IsAngle0=0  IrAngle0=0
      settings: SourceProductBaseCode=PS
  Line 203 : spsDistributedParametersLineLib/Distributed Parameters Line  Phases=3  Length=1.7101  Frequency=50  Resistance=[0.646656091154803 0.0486237908083191 0.0486712220507153;0.0486237908083191 0.646561225344642 0.0486237934466192;0.0486712220507153 0.0486237934466192 0.646656091154803]  Inductance=[0.00282448912315926 0.00133270803418135 0.00132951476746136;0.00133270803418135 0.00282479813276775 0.00133799988507366;0.00132951476746136 0.00133799988507366 0.00282448912315926]  Capacitance=[7.89543174552926e-09 -1.85986777702161e-09 -1.7901190036642e-09;-1.85986777702161e-09 7.82540023894543e-09 -1.8957321828871e-09;-1.7901190036642e-09 -1.8957321828871e-09 7.91264394645417e-09]  x1=[133.233556034884 9752.17913691839 9752.40105493808;314.159265358979 314.159265358979 314.159265358979;1.01113867877432 -0.196177978106079 -1.76715042918016]  x2=[133.241605840749 9751.02850566962 9751.24830666734;314.159265358979 314.159265358979 314.159265358979;1.01124273653415 -0.19637310142644 -1.76734481025143]  x3=[0.121358226101735 23.1805223585639 23.3707533017982;314.159265358979 314.159265358979 314.159265358979;1.00502185987919 -0.223274417371893 -1.79409122574256]  x4=[0.111439643119546 26.3709678368744 26.5615572614046;314.159265358979 314.159265358979 314.159265358979;1.01521912358362 -0.174466214119953 -1.74555454078678]  x5=8.19389748583632e-06  V1=ones(3,3)  V2=ones(3,3)  I1=ones(3,3)  I2=ones(3,3)  nHarmo=1  Measurements=None  Decoupling=off  VsMag0=0  VrMag0=0  VsAngle0=0  VrAngle0=0  IsMag0=0  IrMag0=0  IsAngle0=0  IrAngle0=0
      settings: SourceProductBaseCode=PS
  Line 204 : spsDistributedParametersLineLib/Distributed Parameters Line  Phases=3  Length=0.02  Frequency=50  Resistance=[0.646656091154803 0.0486237908083191 0.0486712220507153;0.0486237908083191 0.646561225344642 0.0486237934466192;0.0486712220507153 0.0486237934466192 0.646656091154803]  Inductance=[0.00282448912315926 0.00133270803418135 0.00132951476746136;0.00133270803418135 0.00282479813276775 0.00133799988507366;0.00132951476746136 0.00133799988507366 0.00282448912315926]  Capacitance=[7.89543174552926e-09 -1.85986777702161e-09 -1.7901190036642e-09;-1.85986777702161e-09 7.82540023894543e-09 -1.8957321828871e-09;-1.7901190036642e-09 -1.8957321828871e-09 7.91264394645417e-09]  x1=[133.233556034884 9752.17913691839 9752.40105493808;314.159265358979 314.159265358979 314.159265358979;1.01368276187795 -0.194156871170561 -1.76512739829396]  x2=[133.233638293661 9752.16721845089 9752.38916167325;314.159265358979 314.159265358979 314.159265358979;1.01368296421427 -0.194157009368751 -1.7651275326431]  x3=[0.118031147757876 24.1503250071093 24.3412069369859;314.159265358979 314.159265358979 314.159265358979;0.999013194242572 -0.177001365688032 -1.74811074712782]  x4=[0.11497385262037 25.4918927464722 25.6833113083434;314.159265358979 314.159265358979 314.159265358979;1.02871213844889 -0.210432870417183 -1.78127819505868]  x5=9.5829454252223e-08  V1=ones(3,3)  V2=ones(3,3)  I1=ones(3,3)  I2=ones(3,3)  nHarmo=1  Measurements=None  Decoupling=off  VsMag0=0  VrMag0=0  VsAngle0=0  VrAngle0=0  IsMag0=0  IrMag0=0  IsAngle0=0  IrAngle0=0
      settings: SourceProductBaseCode=PS
  Line 205 : spsDistributedParametersLineLib/Distributed Parameters Line  Phases=3  Length=0.02  Frequency=50  Resistance=[0.646656091154803 0.0486237908083191 0.0486712220507153;0.0486237908083191 0.646561225344642 0.0486237934466192;0.0486712220507153 0.0486237934466192 0.646656091154803]  Inductance=[0.00282448912315926 0.00133270803418135 0.00132951476746136;0.00133270803418135 0.00282479813276775 0.00133799988507366;0.00132951476746136 0.00133799988507366 0.00282448912315926]  Capacitance=[7.89543174552926e-09 -1.85986777702161e-09 -1.7901190036642e-09;-1.85986777702161e-09 7.82540023894543e-09 -1.8957321828871e-09;-1.7901190036642e-09 -1.8957321828871e-09 7.91264394645417e-09]  x1=[132.809449296114 9777.81056053905 9777.20984376857;314.159265358979 314.159265358979 314.159265358979;1.06968142219943 2.25663427460437 -2.45550101802585]  x2=[132.809514434858 9777.79660369138 9777.19591717147;314.159265358979 314.159265358979 314.159265358979;1.06968200558866 2.25663412662747 -2.45550116072615]  x3=[0.118706563817931 24.1076162546911 24.2971859381218;314.159265358979 314.159265358979 314.159265358979;1.06312202358591 2.2770435731759 -2.43523921175699]  x4=[0.113536321686159 25.6678691156875 25.8573766937651;314.159265358979 314.159265358979 314.159265358979;1.07650933440676 2.23744240365781 -2.47456346422379]  x5=9.5829454252223e-08  V1=ones(3,3)  V2=ones(3,3)  I1=ones(3,3)  I2=ones(3,3)  nHarmo=1  Measurements=None  Decoupling=off  VsMag0=0  VrMag0=0  VsAngle0=0  VrAngle0=0  IsMag0=0  IrMag0=0  IsAngle0=0  IrAngle0=0
      settings: SourceProductBaseCode=PS
  Line 21 : spsDistributedParametersLineLib/Distributed Parameters Line  Phases=3  Length=0.5  Frequency=50  Resistance=[0.646656091154803 0.0486237908083191 0.0486712220507153;0.0486237908083191 0.646561225344642 0.0486237934466192;0.0486712220507153 0.0486237934466192 0.646656091154803]  Inductance=[0.00282448912315926 0.00133270803418135 0.00132951476746136;0.00133270803418135 0.00282479813276775 0.00133799988507366;0.00132951476746136 0.00133799988507366 0.00282448912315926]  Capacitance=[7.89543174552926e-09 -1.85986777702161e-09 -1.7901190036642e-09;-1.85986777702161e-09 7.82540023894543e-09 -1.8957321828871e-09;-1.7901190036642e-09 -1.8957321828871e-09 7.91264394645417e-09]  x1=[131.596700697852 9865.0396113672 9864.44666399304;314.159265358979 314.159265358979 314.159265358979;1.06881002606249 2.2597947814829 -2.45235948559525]  x2=[131.672741119116 9858.70653543795 9858.14819692635;314.159265358979 314.159265358979 314.159265358979;1.06895244845294 2.25940924453326 -2.45273964464847]  x3=[0.178406915299944 6.30879981705719 6.57781757351051;314.159265358979 314.159265358979 314.159265358979;0.686287267891504 2.65451209106245 -2.07467898955589]  x4=[0.0927392416103666 44.4101177944287 44.5015570988937;314.159265358979 314.159265358979 314.159265358979;1.86873666446385 2.20458337318819 -2.50745072977313]  x5=2.39573635630557e-06  V1=ones(3,3)  V2=ones(3,3)  I1=ones(3,3)  I2=ones(3,3)  nHarmo=1  Measurements=None  Decoupling=off  VsMag0=0  VrMag0=0  VsAngle0=0  VrAngle0=0  IsMag0=0  IrMag0=0  IsAngle0=0  IrAngle0=0
      settings: SourceProductBaseCode=PS
  Line 22 : spsDistributedParametersLineLib/Distributed Parameters Line  Phases=3  Length=0.23  Frequency=50  Resistance=[0.646656091154803 0.0486237908083191 0.0486712220507153;0.0486237908083191 0.646561225344642 0.0486237934466192;0.0486712220507153 0.0486237934466192 0.646656091154803]  Inductance=[0.00282448912315926 0.00133270803418135 0.00132951476746136;0.00133270803418135 0.00282479813276775 0.00133799988507366;0.00132951476746136 0.00133799988507366 0.00282448912315926]  Capacitance=[7.89543174552926e-09 -1.85986777702161e-09 -1.7901190036642e-09;-1.85986777702161e-09 7.82540023894543e-09 -1.8957321828871e-09;-1.7901190036642e-09 -1.8957321828871e-09 7.91264394645417e-09]  x1=[131.561022768389 9868.225475962 9867.61640558581;314.159265358979 314.159265358979 314.159265358979;1.06913477528117 2.26030978307765 -2.45184677764775]  x2=[131.596700697851 9865.0396113672 9864.44666399304;314.159265358979 314.159265358979 314.159265358979;1.06921645316029 2.26011766111877 -2.45203629860083]  x3=[0.183021191194099 4.92074574243104 5.16487638300345;314.159265358979 314.159265358979 314.159265358979;0.699530078766377 2.84916653039249 -1.89422739268404]  x4=[0.0888576978788153 46.195452662628 46.2872116549598;314.159265358979 314.159265358979 314.159265358979;1.90775536600978 2.20085849009736 -2.51118183428988]  x5=1.10203872390056e-06  V1=ones(3,3)  V2=ones(3,3)  I1=ones(3,3)  I2=ones(3,3)  nHarmo=1  Measurements=None  Decoupling=off  VsMag0=0  VrMag0=0  VsAngle0=0  VrAngle0=0  IsMag0=0  IrMag0=0  IsAngle0=0  IrAngle0=0
      settings: SourceProductBaseCode=PS
  Line 23 : spsDistributedParametersLineLib/Distributed Parameters Line  Phases=3  Length=1.62  Frequency=50  Resistance=[0.80718830189013 0.0486237908083191 0.0486712220507153;0.0486237908083191 0.807093436079969 0.0486237934466192;0.0486712220507153 0.0486237934466192 0.80718830189013]  Inductance=[0.00279786707424938 0.00133270803418135 0.00132951476746136;0.00133270803418135 0.00279817608385787 0.00133799988507366;0.00132951476746136 0.00133799988507366 0.00279786707424938]  Capacitance=[7.73340098830622e-09 -1.79942827973291e-09 -1.73218055098733e-09;-1.79942827973291e-09 7.66505189233746e-09 -1.83375898618858e-09;-1.73218055098733e-09 -1.83375898618858e-09 7.749673531177e-09]  x1=[54.4938840142718 9868.30989223234 9867.7788132504;314.159265358979 314.159265358979 314.159265358979;1.01985027779978 2.26299862266407 -2.44919829337705]  x2=[54.4941938677022 9868.31273538074 9867.78171404334;314.159265358979 314.159265358979 314.159265358979;1.01985103200153 2.26299572123773 -2.44920121480186]  x3=[0.0475018989148529 24.9830323151725 25.1717342145627;314.159265358979 314.159265358979 314.159265358979;1.0169323416271 2.26132781204967 -2.45087233312526]  x4=[0.0473868696138962 25.0003010564155 25.1890023831144;314.159265358979 314.159265358979 314.159265358979;1.02035192696002 2.26276650507504 -2.44942881569415]  x5=7.70442045759223e-06  V1=ones(3,3)  V2=ones(3,3)  I1=ones(3,3)  I2=ones(3,3)  nHarmo=1  Measurements=None  Decoupling=off  VsMag0=0  VrMag0=0  VsAngle0=0  VrAngle0=0  IsMag0=0  IrMag0=0  IsAngle0=0  IrAngle0=0
      settings: SourceProductBaseCode=PS
  Line 24 : spsDistributedParametersLineLib/Distributed Parameters Line  Phases=3  Length=0.54002  Frequency=50  Resistance=[0.646656091154803 0.0486237908083191 0.0486712220507153;0.0486237908083191 0.646561225344642 0.0486237934466192;0.0486712220507153 0.0486237934466192 0.646656091154803]  Inductance=[0.00282448912315926 0.00133270803418135 0.00132951476746136;0.00133270803418135 0.00282479813276775 0.00133799988507366;0.00132951476746136 0.00133799988507366 0.00282448912315926]  Capacitance=[7.89543174552926e-09 -1.85986777702161e-09 -1.7901190036642e-09;-1.85986777702161e-09 7.82540023894543e-09 -1.8957321828871e-09;-1.7901190036642e-09 -1.8957321828871e-09 7.91264394645417e-09]  x1=[131.476930496598 9875.69630010869 9875.04930166949;314.159265358979 314.159265358979 314.159265358979;1.06847700595697 2.26039161176221 -2.45177138527889]  x2=[131.561022768389 9868.225475962 9867.61640558581;314.159265358979 314.159265358979 314.159265358979;1.06866810665577 2.25993904550464 -2.45221786813668]  x3=[0.183094830693704 4.90000996370689 5.14510680558685;314.159265358979 314.159265358979 314.159265358979;0.69697984456317 2.84004324664083 -1.90314935911359]  x4=[0.0890323477736353 46.1951890945025 46.2868039748363;314.159265358979 314.159265358979 314.159265358979;1.91010414820158 2.20166190235234 -2.51037198715974]  x5=2.58749109426427e-06  V1=ones(3,3)  V2=ones(3,3)  I1=ones(3,3)  I2=ones(3,3)  nHarmo=1  Measurements=None  Decoupling=off  VsMag0=0  VrMag0=0  VsAngle0=0  VrAngle0=0  IsMag0=0  IrMag0=0  IsAngle0=0  IrAngle0=0
      settings: SourceProductBaseCode=PS
  Line 25 : spsDistributedParametersLineLib/Distributed Parameters Line  Phases=3  Length=0.13998  Frequency=50  Resistance=[0.646656091154803 0.0486237908083191 0.0486712220507153;0.0486237908083191 0.646561225344642 0.0486237934466192;0.0486712220507153 0.0486237934466192 0.646656091154803]  Inductance=[0.00282448912315926 0.00133270803418135 0.00132951476746136;0.00133270803418135 0.00282479813276775 0.00133799988507366;0.00132951476746136 0.00133799988507366 0.00282448912315926]  Capacitance=[7.89543174552926e-09 -1.85986777702161e-09 -1.7901190036642e-09;-1.85986777702161e-09 7.82540023894543e-09 -1.8957321828871e-09;-1.7901190036642e-09 -1.8957321828871e-09 7.91264394645417e-09]  x1=[131.476930496598 9875.69630010869 9875.04930166949;314.159265358979 314.159265358979 314.159265358979;1.06907918038734 2.26086999979752 -2.45129254185204]  x2=[131.477737666352 9875.50707139839 9874.86042652478;314.159265358979 314.159265358979 314.159265358979;1.06908783827284 2.26086630362998 -2.4512961631014]  x3=[0.120152634227203 23.5336605418468 23.7248957741594;314.159265358979 314.159265358979 314.159265358979;1.05976922812522 2.29600726586965 -2.41641610588423]  x4=[0.109752830874327 26.7503934941361 26.9416073941244;314.159265358979 314.159265358979 314.159265358979;1.07905971050067 2.22979862357389 -2.48216443842075]  x5=6.70710350311308e-07  V1=ones(3,3)  V2=ones(3,3)  I1=ones(3,3)  I2=ones(3,3)  nHarmo=1  Measurements=None  Decoupling=off  VsMag0=0  VrMag0=0  VsAngle0=0  VrAngle0=0  IsMag0=0  IrMag0=0  IsAngle0=0  IrAngle0=0
      settings: SourceProductBaseCode=PS
  Line 26 : spsDistributedParametersLineLib/Distributed Parameters Line  Phases=3  Length=0.14997  Frequency=50  Resistance=[0.476003738225748 0.351747138225748 0.351747138225748;0.351747138225748 0.476003738225748 0.351747138225748;0.351747138225748 0.351747138225748 0.476003738225748]  Inductance=[0.000705954362986426 0.000459934243504405 0.000459934243504405;0.000459934243504405 0.000705954362986426 0.000459934243504405;0.000459934243504405 0.000459934243504405 0.000705954362986426]  Capacitance=[5.7561313269996e-07 -1.37543883484145e-07 -1.37543912800485e-07;-1.37543883484145e-07 5.75613027339387e-07 -1.37543875208088e-07;-1.37543912800485e-07 -1.37543875208088e-07 5.75613005057695e-07]  x1=[3.00077055114673 9876.59102374936 9876.72098441275;314.159265358979 314.159265358979 314.159265358979;1.26263296644611 2.17876316828644 -2.53355525644402]  x2=[3.00077217372893 9876.54947742322 9876.67943753963;314.159265358979 314.159265358979 314.159265358979;1.2626317114107 2.17876316092323 -2.53355526380719]  x3=[0.0407242629267137 529.750565015631 529.757494666966;314.159265358979 314.159265358979 314.159265358979;1.26159018470407 2.18033137722916 -2.53198704728448]  x4=[0.0407243414040032 532.965919131387 532.972891092363;314.159265358979 314.159265358979 314.159265358979;1.26263243326869 2.17658207101816 -2.53573635387889]  x5=3.31498451375949e-06  V1=ones(3,3)  V2=ones(3,3)  I1=ones(3,3)  I2=ones(3,3)  nHarmo=1  Measurements=None  Decoupling=off  VsMag0=0  VrMag0=0  VsAngle0=0  VrAngle0=0  IsMag0=0  IrMag0=0  IsAngle0=0  IrAngle0=0
      settings: SourceProductBaseCode=PS
  Line 27 : spsDistributedParametersLineLib/Distributed Parameters Line  Phases=3  Length=0.50001  Frequency=50  Resistance=[0.646656091154803 0.0486237908083191 0.0486712220507153;0.0486237908083191 0.646561225344642 0.0486237934466192;0.0486712220507153 0.0486237934466192 0.646656091154803]  Inductance=[0.00282448912315926 0.00133270803418135 0.00132951476746136;0.00133270803418135 0.00282479813276775 0.00133799988507366;0.00132951476746136 0.00133799988507366 0.00282448912315926]  Capacitance=[7.89543174552926e-09 -1.85986777702161e-09 -1.7901190036642e-09;-1.85986777702161e-09 7.82540023894543e-09 -1.8957321828871e-09;-1.7901190036642e-09 -1.8957321828871e-09 7.91264394645417e-09]  x1=[131.396102581756 9883.28723137836 9882.60379428555;314.159265358979 314.159265358979 314.159265358979;1.06832941145038 2.26087158354127 -2.4512972517946]  x2=[131.476930496598 9875.69630010869 9875.04930166949;314.159265358979 314.159265358979 314.159265358979;1.06853723243172 2.26043945774084 -2.45172349375427]  x3=[0.18832457275665 4.31238574258619 4.48747823757262;314.159265358979 314.159265358979 314.159265358979;0.700848394022008 -3.07331896938389 -1.55500119437532]  x4=[0.0865371245803109 47.8741922218531 47.9657863536814;314.159265358979 314.159265358979 314.159265358979;1.96478879728784 2.18704622046569 -2.52497366542852]  x5=2.3957842710327e-06  V1=ones(3,3)  V2=ones(3,3)  I1=ones(3,3)  I2=ones(3,3)  nHarmo=1  Measurements=None  Decoupling=off  VsMag0=0  VrMag0=0  VsAngle0=0  VrAngle0=0  IsMag0=0  IrMag0=0  IsAngle0=0  IrAngle0=0
      settings: SourceProductBaseCode=PS
  Line 28 : spsDistributedParametersLineLib/Distributed Parameters Line  Phases=3  Length=0.17  Frequency=50  Resistance=[0.646656091154803 0.0486237908083191 0.0486712220507153;0.0486237908083191 0.646561225344642 0.0486237934466192;0.0486712220507153 0.0486237934466192 0.646656091154803]  Inductance=[0.00282448912315926 0.00133270803418135 0.00132951476746136;0.00133270803418135 0.00282479813276775 0.00133799988507366;0.00132951476746136 0.00133799988507366 0.00282448912315926]  Capacitance=[7.89543174552926e-09 -1.85986777702161e-09 -1.7901190036642e-09;-1.85986777702161e-09 7.82540023894543e-09 -1.8957321828871e-09;-1.7901190036642e-09 -1.8957321828871e-09 7.91264394645417e-09]  x1=[131.396102581756 9883.28723137836 9882.60379428555;314.159265358979 314.159265358979 314.159265358979;1.06882617073388 2.26126622616584 -2.4509022334982]  x2=[131.396647425564 9883.17004965991 9882.48686600782;314.159265358979 314.159265358979 314.159265358979;1.06883116360746 2.26126490869433 -2.45090350712418]  x3=[0.117444020365948 24.3768685103049 24.5682279957405;314.159265358979 314.159265358979 314.159265358979;1.06227630753233 2.28089022744514 -2.43142134703423]  x4=[0.112310812196159 25.9260402570656 26.1173276976398;314.159265358979 314.159265358979 314.159265358979;1.07541875553123 2.24261645554238 -2.4694262146804]  x5=8.14550361143895e-07  V1=ones(3,3)  V2=ones(3,3)  I1=ones(3,3)  I2=ones(3,3)  nHarmo=1  Measurements=None  Decoupling=off  VsMag0=0  VrMag0=0  VsAngle0=0  VrAngle0=0  IsMag0=0  IrMag0=0  IsAngle0=0  IrAngle0=0
      settings: SourceProductBaseCode=PS
  Line 29 : spsDistributedParametersLineLib/Distributed Parameters Line  Phases=3  Length=0.27999  Frequency=50  Resistance=[0.646656091154803 0.0486237908083191 0.0486712220507153;0.0486237908083191 0.646561225344642 0.0486237934466192;0.0486712220507153 0.0486237934466192 0.646656091154803]  Inductance=[0.00282448912315926 0.00133270803418135 0.00132951476746136;0.00133270803418135 0.00282479813276775 0.00133799988507366;0.00132951476746136 0.00133799988507366 0.00282448912315926]  Capacitance=[7.89543174552926e-09 -1.85986777702161e-09 -1.7901190036642e-09;-1.85986777702161e-09 7.82540023894543e-09 -1.8957321828871e-09;-1.7901190036642e-09 -1.8957321828871e-09 7.91264394645417e-09]  x1=[131.349907125397 9887.72984586618 9887.02556132428;314.159265358979 314.159265358979 314.159265358979;1.06853602239049 2.26137878777284 -2.45079315662409]  x2=[131.396102581757 9883.28723137836 9882.60379428555;314.159265358979 314.159265358979 314.159265358979;1.06866060437652 2.26113469456899 -2.45103389030381]  x3=[0.190998430122671 4.3498499495113 4.47450214150369;314.159265358979 314.159265358979 314.159265358979;0.701874441353109 -2.86555485810355 -1.35406169418671]  x4=[0.0855876694610721 48.7111701410864 48.8028426233765;314.159265358979 314.159265358979 314.159265358979;1.99522551342316 2.17925242158281 -2.5327581429881]  x5=1.341564444804e-06  V1=ones(3,3)  V2=ones(3,3)  I1=ones(3,3)  I2=ones(3,3)  nHarmo=1  Measurements=None  Decoupling=off  VsMag0=0  VrMag0=0  VsAngle0=0  VrAngle0=0  IsMag0=0  IrMag0=0  IsAngle0=0  IrAngle0=0
      settings: SourceProductBaseCode=PS
  Line 3 : spsDistributedParametersLineLib/Distributed Parameters Line  Phases=3  Length=0.03  Frequency=50  Resistance=[0.476003738225748 0.351747138225748 0.351747138225748;0.351747138225748 0.476003738225748 0.351747138225748;0.351747138225748 0.351747138225748 0.476003738225748]  Inductance=[0.000705954362986426 0.000459934243504405 0.000459934243504405;0.000459934243504405 0.000705954362986426 0.000459934243504405;0.000459934243504405 0.000459934243504405 0.000705954362986426]  Capacitance=[5.7561313269996e-07 -1.37543883484145e-07 -1.37543912800485e-07;-1.37543883484145e-07 5.75613027339387e-07 -1.37543875208088e-07;-1.37543912800485e-07 -1.37543875208088e-07 5.75613005057695e-07]  x1=[3.80334430622162 9843.2740131217 9843.523656068;314.159265358979 314.159265358979 314.159265358979;1.32169145669344 2.17729334010131 -2.53499825463759]  x2=[3.80334726356873 9843.27416917428 9843.52381304475;314.159265358979 314.159265358979 314.159265358979;1.32168843955697 2.17729331458677 -2.53499828024873]  x3=[0.0516438066951531 529.884782427987 529.898243946554;314.159265358979 314.159265358979 314.159265358979;1.31571054922321 2.17710382099028 -2.53518832964627]  x4=[0.0517395151506378 529.884846047731 529.898180382787;314.159265358979 314.159265358979 314.159265358979;1.32745013693539 2.17735798878277 -2.53493305011489]  x5=6.63129528657629e-07  V1=ones(3,3)  V2=ones(3,3)  I1=ones(3,3)  I2=ones(3,3)  nHarmo=1  Measurements=None  Decoupling=off  VsMag0=0  VrMag0=0  VsAngle0=0  VrAngle0=0  IsMag0=0  IrMag0=0  IsAngle0=0  IrAngle0=0
      settings: SourceProductBaseCode=PS
  Line 30 : spsDistributedParametersLineLib/Distributed Parameters Line  Phases=3  Length=1.11  Frequency=50  Resistance=[0.502970710632245 0.0486237908083191 0.0486712220507153;0.0486237908083191 0.502875844822084 0.0486237934466192;0.0486712220507153 0.0486237934466192 0.502970710632245]  Inductance=[0.00286900545038753 0.00133270803418135 0.00132951476746136;0.00133270803418135 0.00286931445999602 0.00133799988507366;0.00132951476746136 0.00133799988507366 0.00286900545038753]  Capacitance=[8.11484299003193e-09 -1.94249816214699e-09 -1.86930692621136e-09;-1.94249816214699e-09 8.0425699231653e-09 -1.98049571960044e-09;-1.86930692621136e-09 -1.98049571960044e-09 8.13337738722527e-09]  x1=[236.079077304945 9776.48671476631 9775.73354751084;314.159265358979 314.159265358979 314.159265358979;1.07983361995386 2.24894963292542 -2.46316241605022]  x2=[236.079413902172 9776.49585731864 9775.74270994664;314.159265358979 314.159265358979 314.159265358979;1.07983312774241 2.24894875512332 -2.46316330141347]  x3=[0.206968850170541 24.8692715233504 25.0582939380927;314.159265358979 314.159265358979 314.159265358979;1.07814471752936 2.24758159993277 -2.46453199189806]  x4=[0.206968850203623 24.8692715308017 25.0582939456973;314.159265358979 314.159265358979 314.159265358979;1.07983312772687 2.24894875512376 -2.46316330141309]  x5=5.37516004033389e-06  V1=ones(3,3)  V2=ones(3,3)  I1=ones(3,3)  I2=ones(3,3)  nHarmo=1  Measurements=None  Decoupling=off  VsMag0=0  VrMag0=0  VsAngle0=0  VrAngle0=0  IsMag0=0  IrMag0=0  IsAngle0=0  IrAngle0=0
      settings: SourceProductBaseCode=PS
  Line 31 : spsDistributedParametersLineLib/Distributed Parameters Line  Phases=3  Length=0.02  Frequency=50  Resistance=[0.646656091154803 0.0486237908083191 0.0486712220507153;0.0486237908083191 0.646561225344642 0.0486237934466192;0.0486712220507153 0.0486237934466192 0.646656091154803]  Inductance=[0.00282448912315926 0.00133270803418135 0.00132951476746136;0.00133270803418135 0.00282479813276775 0.00133799988507366;0.00132951476746136 0.00133799988507366 0.00282448912315926]  Capacitance=[7.89543174552926e-09 -1.85986777702161e-09 -1.7901190036642e-09;-1.85986777702161e-09 7.82540023894543e-09 -1.8957321828871e-09;-1.7901190036642e-09 -1.8957321828871e-09 7.91264394645417e-09]  x1=[132.809332030151 9777.83927933201 9777.23853078397;314.159265358979 314.159265358979 314.159265358979;1.06967986790278 2.25663575440883 -2.45549955085789]  x2=[132.809449296114 9777.81056053905 9777.20984376857;314.159265358979 314.159265358979 314.159265358979;1.06968142219942 2.25663427460437 -2.45550101802585]  x3=[0.12241394898276 22.8142750283999 23.0036735462151;314.159265358979 314.159265358979 314.159265358979;1.06401544033668 2.27498423682034 -2.43731489487654]  x4=[0.109827708627678 26.9586712424282 27.148348981877;314.159265358979 314.159265358979 314.159265358979;1.07596325832956 2.24108481420619 -2.47093122529088]  x5=9.5829454252223e-08  V1=ones(3,3)  V2=ones(3,3)  I1=ones(3,3)  I2=ones(3,3)  nHarmo=1  Measurements=None  Decoupling=off  VsMag0=0  VrMag0=0  VsAngle0=0  VrAngle0=0  IsMag0=0  IrMag0=0  IsAngle0=0  IrAngle0=0
      settings: SourceProductBaseCode=PS
  Line 32 : spsDistributedParametersLineLib/Distributed Parameters Line  Phases=3  Length=1.15  Frequency=50  Resistance=[0.646656091154803 0.0486237908083191 0.0486712220507153;0.0486237908083191 0.646561225344642 0.0486237934466192;0.0486712220507153 0.0486237934466192 0.646656091154803]  Inductance=[0.00282448912315926 0.00133270803418135 0.00132951476746136;0.00133270803418135 0.00282479813276775 0.00133799988507366;0.00132951476746136 0.00133799988507366 0.00282448912315926]  Capacitance=[7.89543174552926e-09 -1.85986777702161e-09 -1.7901190036642e-09;-1.85986777702161e-09 7.82540023894543e-09 -1.8957321828871e-09;-1.7901190036642e-09 -1.8957321828871e-09 7.91264394645417e-09]  x1=[132.809332030151 9777.83927933201 9777.23853078397;314.159265358979 314.159265358979 314.159265358979;1.06797889523424 2.25528444334018 -2.45685214827899]  x2=[132.814920717303 9776.70813842728 9776.1095975772;314.159265358979 314.159265358979 314.159265358979;1.0680295016704 2.2552567255705 -2.45687943462532]  x3=[0.119948699668048 23.6496171606434 23.8386637570523;314.159265358979 314.159265358979 314.159265358979;1.05759397079875 2.27803907823479 -2.43428815050954]  x4=[0.11217727126065 26.0617229660094 26.2507295797827;314.159265358979 314.159265358979 314.159265358979;1.07734427470346 2.23329758183875 -2.47868240896714]  x5=5.51019361950282e-06  V1=ones(3,3)  V2=ones(3,3)  I1=ones(3,3)  I2=ones(3,3)  nHarmo=1  Measurements=None  Decoupling=off  VsMag0=0  VrMag0=0  VsAngle0=0  VrAngle0=0  IsMag0=0  IrMag0=0  IsAngle0=0  IrAngle0=0
      settings: SourceProductBaseCode=PS
  Line 33 : spsDistributedParametersLineLib/Distributed Parameters Line  Phases=3  Length=0.18999  Frequency=50  Resistance=[0.646656091154803 0.0486237908083191 0.0486712220507153;0.0486237908083191 0.646561225344642 0.0486237934466192;0.0486712220507153 0.0486237934466192 0.646656091154803]  Inductance=[0.00282448912315926 0.00133270803418135 0.00132951476746136;0.00133270803418135 0.00282479813276775 0.00133799988507366;0.00132951476746136 0.00133799988507366 0.00282448912315926]  Capacitance=[7.89543174552926e-09 -1.85986777702161e-09 -1.7901190036642e-09;-1.85986777702161e-09 7.82540023894543e-09 -1.8957321828871e-09;-1.7901190036642e-09 -1.8957321828871e-09 7.91264394645417e-09]  x1=[132.814920717304 9776.70813842728 9776.1095975772;314.159265358979 314.159265358979 314.159265358979;1.06947459084874 2.25640475401211 -2.45573031334193]  x2=[132.815267440374 9776.62309105432 9776.02469674343;314.159265358979 314.159265358979 314.159265358979;1.06947857744133 2.25640266892325 -2.45573236361278]  x3=[0.11786466753466 24.326601633631 24.5160715163124;314.159265358979 314.159265358979 314.159265358979;1.06674471120088 2.2666805046448 -2.44552811782658]  x4=[0.114364415439566 25.4262626882038 25.6157370072646;314.159265358979 314.159265358979 314.159265358979;1.07200169450163 2.24634909209699 -2.46571907806452]  x5=9.10331900668992e-07  V1=ones(3,3)  V2=ones(3,3)  I1=ones(3,3)  I2=ones(3,3)  nHarmo=1  Measurements=None  Decoupling=off  VsMag0=0  VrMag0=0  VsAngle0=0  VrAngle0=0  IsMag0=0  IrMag0=0  IsAngle0=0  IrAngle0=0
      settings: SourceProductBaseCode=PS
  Line 34 : spsDistributedParametersLineLib/Distributed Parameters Line  Phases=3  Length=0.34002  Frequency=50  Resistance=[0.646656091154803 0.0486237908083191 0.0486712220507153;0.0486237908083191 0.646561225344642 0.0486237934466192;0.0486712220507153 0.0486237934466192 0.646656091154803]  Inductance=[0.00282448912315926 0.00133270803418135 0.00132951476746136;0.00133270803418135 0.00282479813276775 0.00133799988507366;0.00132951476746136 0.00133799988507366 0.00282448912315926]  Capacitance=[7.89543174552926e-09 -1.85986777702161e-09 -1.7901190036642e-09;-1.85986777702161e-09 7.82540023894543e-09 -1.8957321828871e-09;-1.7901190036642e-09 -1.8957321828871e-09 7.91264394645417e-09]  x1=[132.814920717304 9776.70813842728 9776.1095975772;314.159265358979 314.159265358979 314.159265358979;1.06924875285806 2.25622534056111 -2.45590989758183]  x2=[132.815866703899 9776.52190926233 9775.92375150461;314.159265358979 314.159265358979 314.159265358979;1.06925685933794 2.25622139552165 -2.45591377295975]  x3=[0.118245912731593 24.214860651153 24.4042721818858;314.159265358979 314.159265358979 314.159265358979;1.06313074276336 2.26955055595705 -2.44269177030435]  x4=[0.113970080502887 25.5309799330117 25.7203641577214;314.159265358979 314.159265358979 314.159265358979;1.07508309734617 2.24318705071361 -2.46885204001027]  x5=1.62919655174204e-06  V1=ones(3,3)  V2=ones(3,3)  I1=ones(3,3)  I2=ones(3,3)  nHarmo=1  Measurements=None  Decoupling=off  VsMag0=0  VrMag0=0  VsAngle0=0  VrAngle0=0  IsMag0=0  IrMag0=0  IsAngle0=0  IrAngle0=0
      settings: SourceProductBaseCode=PS
  Line 35 : spsDistributedParametersLineLib/Distributed Parameters Line  Phases=3  Length=0.12001  Frequency=50  Resistance=[0.646656091154803 0.0486237908083191 0.0486712220507153;0.0486237908083191 0.646561225344642 0.0486237934466192;0.0486712220507153 0.0486237934466192 0.646656091154803]  Inductance=[0.00282448912315926 0.00133270803418135 0.00132951476746136;0.00133270803418135 0.00282479813276775 0.00133799988507366;0.00132951476746136 0.00133799988507366 0.00282448912315926]  Capacitance=[7.89543174552926e-09 -1.85986777702161e-09 -1.7901190036642e-09;-1.85986777702161e-09 7.82540023894543e-09 -1.8957321828871e-09;-1.7901190036642e-09 -1.8957321828871e-09 7.91264394645417e-09]  x1=[132.815866703899 9776.52190926233 9775.92375150461;314.159265358979 314.159265358979 314.159265358979;1.06958803721122 2.25648449459087 -2.45565042343885]  x2=[132.816049174746 9776.48524055818 9775.88716873147;314.159265358979 314.159265358979 314.159265358979;1.06958949815274 2.25648427350878 -2.45565063116861]  x3=[0.117232453044906 24.5473088239398 24.7368304981344;314.159265358979 314.159265358979 314.159265358979;1.06605962660293 2.26576751748864 -2.44643465677593]  x4=[0.115006649030383 25.2082541553428 25.3977345078221;314.159265358979 314.159265358979 314.159265358979;1.0730038099879 2.24730301662849 -2.46476836236287]  x5=5.75024640240464e-07  V1=ones(3,3)  V2=ones(3,3)  I1=ones(3,3)  I2=ones(3,3)  nHarmo=1  Measurements=None  Decoupling=off  VsMag0=0  VrMag0=0  VsAngle0=0  VrAngle0=0  IsMag0=0  IrMag0=0  IsAngle0=0  IrAngle0=0
      settings: SourceProductBaseCode=PS
  Line 36 : spsDistributedParametersLineLib/Distributed Parameters Line  Phases=3  Length=0.82  Frequency=50  Resistance=[0.646656091154803 0.0486237908083191 0.0486712220507153;0.0486237908083191 0.646561225344642 0.0486237934466192;0.0486712220507153 0.0486237934466192 0.646656091154803]  Inductance=[0.00282448912315926 0.00133270803418135 0.00132951476746136;0.00133270803418135 0.00282479813276775 0.00133799988507366;0.00132951476746136 0.00133799988507366 0.00282448912315926]  Capacitance=[7.89543174552926e-09 -1.85986777702161e-09 -1.7901190036642e-09;-1.85986777702161e-09 7.82540023894543e-09 -1.8957321828871e-09;-1.7901190036642e-09 -1.8957321828871e-09 7.91264394645417e-09]  x1=[132.815866703899 9776.52190926233 9775.92375150461;314.159265358979 314.159265358979 314.159265358979;1.06853435238091 2.25564741119711 -2.45648830367673]  x2=[132.816743364638 9776.3160064176 9775.71817184932;314.159265358979 314.159265358979 314.159265358979;1.06854443249126 2.25564036239935 -2.45649526762545]  x3=[0.117104627695193 24.5294241633692 24.7186220464174;314.159265358979 314.159265358979 314.159265358979;1.06639643190664 2.2599239225563 -2.45224849553761]  x4=[0.115054868156884 25.1844218182697 25.373630478697;314.159265358979 314.159265358979 314.159265358979;1.06947503592072 2.25050701981661 -2.46159470271223]  x5=3.92900762434114e-06  V1=ones(3,3)  V2=ones(3,3)  I1=ones(3,3)  I2=ones(3,3)  nHarmo=1  Measurements=None  Decoupling=off  VsMag0=0  VrMag0=0  VsAngle0=0  VrAngle0=0  IsMag0=0  IrMag0=0  IsAngle0=0  IrAngle0=0
      settings: SourceProductBaseCode=PS
  Line 37 : spsDistributedParametersLineLib/Distributed Parameters Line  Phases=3  Length=1.11  Frequency=50  Resistance=[0.646656091154803 0.0486237908083191 0.0486712220507153;0.0486237908083191 0.646561225344642 0.0486237934466192;0.0486712220507153 0.0486237934466192 0.646656091154803]  Inductance=[0.00282448912315926 0.00133270803418135 0.00132951476746136;0.00133270803418135 0.00282479813276775 0.00133799988507366;0.00132951476746136 0.00133799988507366 0.00282448912315926]  Capacitance=[7.89543174552926e-09 -1.85986777702161e-09 -1.7901190036642e-09;-1.85986777702161e-09 7.82540023894543e-09 -1.8957321828871e-09;-1.7901190036642e-09 -1.8957321828871e-09 7.91264394645417e-09]  x1=[132.797050043835 9780.50733909135 9779.90266205066;314.159265358979 314.159265358979 314.159265358979;1.06790521900017 2.25544342892735 -2.4566942150219]  x2=[132.809332030152 9777.83927933201 9777.23853078397;314.159265358979 314.159265358979 314.159265358979;1.06803910665614 2.25533227736031 -2.45680426872426]  x3=[0.126243122440653 21.600430243079 21.7892603262904;314.159265358979 314.159265358979 314.159265358979;1.05102122648142 2.29821963644025 -2.41432677929264]  x4=[0.105896375579435 28.1465289360051 28.3356091346002;314.159265358979 314.159265358979 314.159265358979;1.0863486643102 2.2213483593583 -2.49054235691166]  x5=5.31853471099837e-06  V1=ones(3,3)  V2=ones(3,3)  I1=ones(3,3)  I2=ones(3,3)  nHarmo=1  Measurements=None  Decoupling=off  VsMag0=0  VrMag0=0  VsAngle0=0  VrAngle0=0  IsMag0=0  IrMag0=0  IsAngle0=0  IrAngle0=0
      settings: SourceProductBaseCode=PS
  Line 38 : spsDistributedParametersLineLib/Distributed Parameters Line  Phases=3  Length=0.21  Frequency=50  Resistance=[0.646656091154803 0.0486237908083191 0.0486712220507153;0.0486237908083191 0.646561225344642 0.0486237934466192;0.0486712220507153 0.0486237934466192 0.646656091154803]  Inductance=[0.00282448912315926 0.00133270803418135 0.00132951476746136;0.00133270803418135 0.00282479813276775 0.00133799988507366;0.00132951476746136 0.00133799988507366 0.00282448912315926]  Capacitance=[7.89543174552926e-09 -1.85986777702161e-09 -1.7901190036642e-09;-1.85986777702161e-09 7.82540023894543e-09 -1.8957321828871e-09;-1.7901190036642e-09 -1.8957321828871e-09 7.91264394645417e-09]  x1=[132.797050043835 9780.50733909135 9779.90266205066;314.159265358979 314.159265358979 314.159265358979;1.06925997599281 2.25651969438026 -2.45561692504048]  x2=[132.796528554894 9780.55740580867 9779.95238560685;314.159265358979 314.159265358979 314.159265358979;1.06926047032597 2.25651318333107 -2.45562343802106]  x3=[0.11573276605365 24.8896574121599 25.0790057083605;314.159265358979 314.159265358979 314.159265358979;1.08018014080533 2.23601506956773 -2.47597155934642]  x4=[0.116475404779802 24.8895109603478 25.0791497652497;314.159265358979 314.159265358979 314.159265358979;1.05809482004708 2.27676677937034 -2.43552030781744]  x5=1.00620926964834e-06  V1=ones(3,3)  V2=ones(3,3)  I1=ones(3,3)  I2=ones(3,3)  nHarmo=1  Measurements=None  Decoupling=off  VsMag0=0  VrMag0=0  VsAngle0=0  VrAngle0=0  IsMag0=0  IrMag0=0  IsAngle0=0  IrAngle0=0
      settings: SourceProductBaseCode=PS
  Line 39 : spsDistributedParametersLineLib/Distributed Parameters Line  Phases=3  Length=0.23002  Frequency=50  Resistance=[0.476003738225748 0.351747138225748 0.351747138225748;0.351747138225748 0.476003738225748 0.351747138225748;0.351747138225748 0.351747138225748 0.476003738225748]  Inductance=[0.000705954362986426 0.000459934243504405 0.000459934243504405;0.000459934243504405 0.000705954362986426 0.000459934243504405;0.000459934243504405 0.000459934243504405 0.000705954362986426]  Capacitance=[5.7561313269996e-07 -1.37543883484145e-07 -1.37543912800485e-07;-1.37543883484145e-07 5.75613027339387e-07 -1.37543875208088e-07;-1.37543912800485e-07 -1.37543875208088e-07 5.75613005057695e-07]  x1=[5.6230599394157 9781.64847033851 9781.76974796652;314.159265358979 314.159265358979 314.159265358979;1.27410285446112 2.17416095990665 -2.53813208003178]  x2=[5.62306711287961 9781.65295127456 9781.77422895746;314.159265358979 314.159265358979 314.159265358979;1.27409990847979 2.17416022343536 -2.53813281650296]  x3=[0.0762387684728777 526.039448277767 526.045929751241;314.159265358979 314.159265358979 314.159265358979;1.27250405812521 2.17320341223594 -2.53908962762858]  x4=[0.076238768479132 526.039448370704 526.045929843336;314.159265358979 314.159265358979 314.159265358979;1.27409990975831 2.17416022343517 -2.53813281650281]  x5=5.08443513939426e-06  V1=ones(3,3)  V2=ones(3,3)  I1=ones(3,3)  I2=ones(3,3)  nHarmo=1  Measurements=None  Decoupling=off  VsMag0=0  VrMag0=0  VsAngle0=0  VrAngle0=0  IsMag0=0  IrMag0=0  IsAngle0=0  IrAngle0=0
      settings: SourceProductBaseCode=PS
  Line 4 : spsDistributedParametersLineLib/Distributed Parameters Line  Phases=3  Length=0.02  Frequency=50  Resistance=[0.646656091154803 0.0486237908083191 0.0486712220507153;0.0486237908083191 0.646561225344642 0.0486237934466192;0.0486712220507153 0.0486237934466192 0.646656091154803]  Inductance=[0.00282448912315926 0.00133270803418135 0.00132951476746136;0.00133270803418135 0.00282479813276775 0.00133799988507366;0.00132951476746136 0.00133799988507366 0.00282448912315926]  Capacitance=[7.89543174552926e-09 -1.85986777702161e-09 -1.7901190036642e-09;-1.85986777702161e-09 7.82540023894543e-09 -1.8957321828871e-09;-1.7901190036642e-09 -1.8957321828871e-09 7.91264394645417e-09]  x1=[131.763809776127 9846.88411593864 9846.39278960383;314.159265358979 314.159265358979 314.159265358979;1.06994459722368 2.25933500524722 -2.45280498745223]  x2=[131.763824950482 9846.88109991893 9846.38978083538;314.159265358979 314.159265358979 314.159265358979;1.0699447160549 2.25933499503049 -2.45280499659224]  x3=[0.115748439228276 24.8989408523263 25.0901491809546;314.159265358979 314.159265358979 314.159265358979;1.06814785374464 2.26403576179389 -2.44813773945037]  x4=[0.114661110967253 25.2189353979901 25.4101245521894;314.159265358979 314.159265358979 314.159265358979;1.07172824942315 2.25467011984188 -2.45743726132294]  x5=9.5829454252223e-08  V1=ones(3,3)  V2=ones(3,3)  I1=ones(3,3)  I2=ones(3,3)  nHarmo=1  Measurements=None  Decoupling=off  VsMag0=0  VrMag0=0  VsAngle0=0  VrAngle0=0  IsMag0=0  IrMag0=0  IsAngle0=0  IrAngle0=0
      settings: SourceProductBaseCode=PS
  Line 40 : spsDistributedParametersLineLib/Distributed Parameters Line  Phases=3  Length=0.24001  Frequency=50  Resistance=[0.646656091154803 0.0486237908083191 0.0486712220507153;0.0486237908083191 0.646561225344642 0.0486237934466192;0.0486712220507153 0.0486237934466192 0.646656091154803]  Inductance=[0.00282448912315926 0.00133270803418135 0.00132951476746136;0.00133270803418135 0.00282479813276775 0.00133799988507366;0.00132951476746136 0.00133799988507366 0.00282448912315926]  Capacitance=[7.89543174552926e-09 -1.85986777702161e-09 -1.7901190036642e-09;-1.85986777702161e-09 7.82540023894543e-09 -1.8957321828871e-09;-1.7901190036642e-09 -1.8957321828871e-09 7.91264394645417e-09]  x1=[132.571645858499 9793.55793368673 9793.59468692091;314.159265358979 314.159265358979 314.159265358979;1.0140711138123 -0.192057889450736 -1.76302197472672]  x2=[132.622916358163 9790.14137890445 9790.19164885648;314.159265358979 314.159265358979 314.159265358979;1.01409473810605 -0.192228304764726 -1.76319271318381]  x3=[0.195968644446998 6.31558895599864 6.36422182206112;314.159265358979 314.159265358979 314.159265358979;0.467378005510713 0.573612126750516 -1.02874405852631]  x4=[0.120511367438203 45.4838735005614 45.6838055419843;314.159265358979 314.159265358979 314.159265358979;2.02072976670096 -0.288686919730652 -1.85675587077033]  x5=1.1500013657538e-06  V1=ones(3,3)  V2=ones(3,3)  I1=ones(3,3)  I2=ones(3,3)  nHarmo=1  Measurements=None  Decoupling=off  VsMag0=0  VrMag0=0  VsAngle0=0  VrAngle0=0  IsMag0=0  IrMag0=0  IsAngle0=0  IrAngle0=0
      settings: SourceProductBaseCode=PS
  Line 41 : spsDistributedParametersLineLib/Distributed Parameters Line  Phases=3  Length=0.24  Frequency=50  Resistance=[0.646656091154803 0.0486237908083191 0.0486712220507153;0.0486237908083191 0.646561225344642 0.0486237934466192;0.0486712220507153 0.0486237934466192 0.646656091154803]  Inductance=[0.00282448912315926 0.00133270803418135 0.00132951476746136;0.00133270803418135 0.00282479813276775 0.00133799988507366;0.00132951476746136 0.00133799988507366 0.00282448912315926]  Capacitance=[7.89543174552926e-09 -1.85986777702161e-09 -1.7901190036642e-09;-1.85986777702161e-09 7.82540023894543e-09 -1.8957321828871e-09;-1.7901190036642e-09 -1.8957321828871e-09 7.91264394645417e-09]  x1=[132.789126266165 9781.02683598407 9780.42031592206;314.159265358979 314.159265358979 314.159265358979;1.06915987448028 2.25651546175168 -2.45562122510455]  x2=[132.797050043832 9780.50733909159 9779.90266205088;314.159265358979 314.159265358979 314.159265358979;1.06921481742648 2.25648381886518 -2.45565283470652]  x3=[0.138294605147496 21.6036323755844 21.7919218611453;314.159265358979 314.159265358979 314.159265358979;0.998464932902589 2.27605556589534 -2.43689570121973]  x4=[0.094736284763423 28.1720995163247 28.3623163256719;314.159265358979 314.159265358979 314.159265358979;1.17207955373526 2.241250111673 -2.47029042679963]  x5=1.14995345102668e-06  V1=ones(3,3)  V2=ones(3,3)  I1=ones(3,3)  I2=ones(3,3)  nHarmo=1  Measurements=None  Decoupling=off  VsMag0=0  VrMag0=0  VsAngle0=0  VrAngle0=0  IsMag0=0  IrMag0=0  IsAngle0=0  IrAngle0=0
      settings: SourceProductBaseCode=PS
  Line 42 : spsDistributedParametersLineLib/Distributed Parameters Line  Phases=3  Length=0.02  Frequency=50  Resistance=[0.646656091154803 0.0486237908083191 0.0486712220507153;0.0486237908083191 0.646561225344642 0.0486237934466192;0.0486712220507153 0.0486237934466192 0.646656091154803]  Inductance=[0.00282448912315926 0.00133270803418135 0.00132951476746136;0.00133270803418135 0.00282479813276775 0.00133799988507366;0.00132951476746136 0.00133799988507366 0.00282448912315926]  Capacitance=[7.89543174552926e-09 -1.85986777702161e-09 -1.7901190036642e-09;-1.85986777702161e-09 7.82540023894543e-09 -1.8957321828871e-09;-1.7901190036642e-09 -1.8957321828871e-09 7.91264394645417e-09]  x1=[132.571645858499 9793.55793368673 9793.59468692091;314.159265358979 314.159265358979 314.159265358979;1.01440229168558 -0.191794790381519 -1.76275862520582]  x2=[132.571691274989 9793.55085497663 9793.58761662274;314.159265358979 314.159265358979 314.159265358979;1.01440253699171 -0.191795110078639 -1.76275894204222]  x3=[0.117189403725893 24.430133204933 24.6215067064136;314.159265358979 314.159265358979 314.159265358979;1.00782771998935 -0.18665928468683 -1.75766792174883]  x4=[0.114637527315984 25.4164056406712 25.6080509559884;314.159265358979 314.159265358979 314.159265358979;1.02109302488817 -0.196754780011776 -1.76767699843456]  x5=9.5829454252223e-08  V1=ones(3,3)  V2=ones(3,3)  I1=ones(3,3)  I2=ones(3,3)  nHarmo=1  Measurements=None  Decoupling=off  VsMag0=0  VrMag0=0  VsAngle0=0  VrAngle0=0  IsMag0=0  IrMag0=0  IsAngle0=0  IrAngle0=0
      settings: SourceProductBaseCode=PS
  Line 43 : spsDistributedParametersLineLib/Distributed Parameters Line  Phases=3  Length=0.5  Frequency=50  Resistance=[0.646656091154803 0.0486237908083191 0.0486712220507153;0.0486237908083191 0.646561225344642 0.0486237934466192;0.0486712220507153 0.0486237934466192 0.646656091154803]  Inductance=[0.00282448912315926 0.00133270803418135 0.00132951476746136;0.00133270803418135 0.00282479813276775 0.00133799988507366;0.00132951476746136 0.00133799988507366 0.00282448912315926]  Capacitance=[7.89543174552926e-09 -1.85986777702161e-09 -1.7901190036642e-09;-1.85986777702161e-09 7.82540023894543e-09 -1.8957321828871e-09;-1.7901190036642e-09 -1.8957321828871e-09 7.91264394645417e-09]  x1=[132.463644567909 9800.85070742944 9800.85908991131;314.159265358979 314.159265358979 314.159265358979;1.01362452835019 -0.19200583747329 -1.76296961325886]  x2=[132.571645858499 9793.55793368673 9793.59468692091;314.159265358979 314.159265358979 314.159265358979;1.01367975462284 -0.192368798623072 -1.76333317986257]  x3=[0.197406279589044 6.06772792911599 6.10255132458703;314.159265358979 314.159265358979 314.159265358979;0.466346338482951 0.642027293605158 -0.962109646703075]  x4=[0.120486541143136 45.9827950150991 46.1825376125341;314.159265358979 314.159265358979 314.159265358979;2.03322751873653 -0.290418522632651 -1.85850838627736]  x5=2.39573635630557e-06  V1=ones(3,3)  V2=ones(3,3)  I1=ones(3,3)  I2=ones(3,3)  nHarmo=1  Measurements=None  Decoupling=off  VsMag0=0  VrMag0=0  VsAngle0=0  VrAngle0=0  IsMag0=0  IrMag0=0  IsAngle0=0  IrAngle0=0
      settings: SourceProductBaseCode=PS
  Line 44 : spsDistributedParametersLineLib/Distributed Parameters Line  Phases=3  Length=1.11  Frequency=50  Resistance=[0.502970710632245 0.0486237908083191 0.0486712220507153;0.0486237908083191 0.502875844822084 0.0486237934466192;0.0486712220507153 0.0486237934466192 0.502970710632245]  Inductance=[0.00286900545038753 0.00133270803418135 0.00132951476746136;0.00133270803418135 0.00286931445999602 0.00133799988507366;0.00132951476746136 0.00133799988507366 0.00286900545038753]  Capacitance=[8.11484299003193e-09 -1.94249816214699e-09 -1.86930692621136e-09;-1.94249816214699e-09 8.0425699231653e-09 -1.98049571960044e-09;-1.86930692621136e-09 -1.98049571960044e-09 8.13337738722527e-09]  x1=[235.854314205501 9837.47042487058 9837.20377657701;314.159265358979 314.159265358979 314.159265358979;0.993194279468019 -0.184885896585883 -1.75587527735441]  x2=[235.854650482287 9837.47962445227 9837.2129966266;314.159265358979 314.159265358979 314.159265358979;0.99319378725628 -0.184886774387986 -1.75587616271766]  x3=[0.206771801930645 25.0244009158736 25.2158615580561;314.159265358979 314.159265358979 314.159265358979;0.991505376943513 -0.186253929578869 -1.75724485320201]  x4=[0.206771802019709 25.0244009233717 25.215861565691;314.159265358979 314.159265358979 314.159265358979;0.993193787351219 -0.184886774387202 -1.7558761627176]  x5=5.37516004033389e-06  V1=ones(3,3)  V2=ones(3,3)  I1=ones(3,3)  I2=ones(3,3)  nHarmo=1  Measurements=None  Decoupling=off  VsMag0=0  VrMag0=0  VsAngle0=0  VrAngle0=0  IsMag0=0  IrMag0=0  IsAngle0=0  IrAngle0=0
      settings: SourceProductBaseCode=PS
  Line 45 : spsDistributedParametersLineLib/Distributed Parameters Line  Phases=3  Length=0.03  Frequency=50  Resistance=[0.476003738225748 0.351747138225748 0.351747138225748;0.351747138225748 0.476003738225748 0.351747138225748;0.351747138225748 0.351747138225748 0.476003738225748]  Inductance=[0.000705954362986426 0.000459934243504405 0.000459934243504405;0.000459934243504405 0.000705954362986426 0.000459934243504405;0.000459934243504405 0.000459934243504405 0.000705954362986426]  Capacitance=[5.7561313269996e-07 -1.37543883484145e-07 -1.37543912800485e-07;-1.37543883484145e-07 5.75613027339387e-07 -1.37543875208088e-07;-1.37543912800485e-07 -1.37543875208088e-07 5.75613005057695e-07]  x1=[4.06113764319374 9838.54539143333 9839.28246477345;314.159265358979 314.159265358979 314.159265358979;1.25934197027703 -0.108222246185315 -1.67903740641506]  x2=[4.06113849494603 9838.54554764787 9839.28262144573;314.159265358979 314.159265358979 314.159265358979;1.25933905933857 -0.10822227168487 -1.67903743204118]  x3=[0.0550936453727556 529.630294037614 529.669867869187;314.159265358979 314.159265358979 314.159265358979;1.25397307408713 -0.108411765214978 -1.67922748150114]  x4=[0.0552966608561192 529.630230503591 529.669931408302;314.159265358979 314.159265358979 314.159265358979;1.26448027999306 -0.108157597538327 -1.67897220186093]  x5=6.63129528657629e-07  V1=ones(3,3)  V2=ones(3,3)  I1=ones(3,3)  I2=ones(3,3)  nHarmo=1  Measurements=None  Decoupling=off  VsMag0=0  VrMag0=0  VsAngle0=0  VrAngle0=0  IsMag0=0  IrMag0=0  IsAngle0=0  IrAngle0=0
      settings: SourceProductBaseCode=PS
  Line 46 : spsDistributedParametersLineLib/Distributed Parameters Line  Phases=3  Length=0.28003  Frequency=50  Resistance=[0.476003738225748 0.351747138225748 0.351747138225748;0.351747138225748 0.476003738225748 0.351747138225748;0.351747138225748 0.351747138225748 0.476003738225748]  Inductance=[0.000705954362986426 0.000459934243504405 0.000459934243504405;0.000459934243504405 0.000705954362986426 0.000459934243504405;0.000459934243504405 0.000459934243504405 0.000705954362986426]  Capacitance=[5.7561313269996e-07 -1.37543883484145e-07 -1.37543912800485e-07;-1.37543883484145e-07 5.75613027339387e-07 -1.37543875208088e-07;-1.37543912800485e-07 -1.37543875208088e-07 5.75613005057695e-07]  x1=[4.06113764319374 9838.54539143333 9839.28246477345;314.159265358979 314.159265358979 314.159265358979;1.2576056929024 -0.109262692990563 -1.68007785313988]  x2=[4.06488389119121 9837.53031252039 9838.2684138264;314.159265358979 314.159265358979 314.159265358979;1.25110932525924 -0.109295686818563 -1.6801112931524]  x3=[0.0795017874211303 503.808062672123 503.810843308063;314.159265358979 314.159265358979 314.159265358979;0.146202409027003 -0.097266533032414 -1.66828947152461]  x4=[0.103029706043435 554.146420218594 554.22037238641;314.159265358979 314.159265358979 314.159265358979;2.01512893297034 -0.121313448930483 -1.6919386928395]  x5=6.18987206366653e-06  V1=ones(3,3)  V2=ones(3,3)  I1=ones(3,3)  I2=ones(3,3)  nHarmo=1  Measurements=None  Decoupling=off  VsMag0=0  VrMag0=0  VsAngle0=0  VrAngle0=0  IsMag0=0  IrMag0=0  IsAngle0=0  IrAngle0=0
      settings: SourceProductBaseCode=PS
  Line 47 : spsDistributedParametersLineLib/Distributed Parameters Line  Phases=3  Length=0.28003  Frequency=50  Resistance=[0.646656091154803 0.0486237908083191 0.0486712220507153;0.0486237908083191 0.646561225344642 0.0486237934466192;0.0486712220507153 0.0486237934466192 0.646656091154803]  Inductance=[0.00282448912315926 0.00133270803418135 0.00132951476746136;0.00133270803418135 0.00282479813276775 0.00133799988507366;0.00132951476746136 0.00133799988507366 0.00282448912315926]  Capacitance=[7.89543174552926e-09 -1.85986777702161e-09 -1.7901190036642e-09;-1.85986777702161e-09 7.82540023894543e-09 -1.8957321828871e-09;-1.7901190036642e-09 -1.8957321828871e-09 7.91264394645417e-09]  x1=[131.974883970949 9836.49372751531 9836.37348162638;314.159265358979 314.159265358979 314.159265358979;1.01361577111541 -0.190116150305535 -1.76107882477881]  x2=[132.042752270136 9831.39156427917 9831.28920891362;314.159265358979 314.159265358979 314.159265358979;1.01366791583491 -0.190340132443455 -1.76130281798942]  x3=[0.211623140526362 6.67388751924019 6.5564352456938;314.159265358979 314.159265358979 314.159265358979;0.447425788740306 1.41051388651929 -0.185818464698286]  x4=[0.124910559079367 50.6785236376165 50.875566928245;314.159265358979 314.159265358979 314.159265358979;2.15320263619403 -0.322409625668031 -1.89058833868094]  x5=1.3417561037125e-06  V1=ones(3,3)  V2=ones(3,3)  I1=ones(3,3)  I2=ones(3,3)  nHarmo=1  Measurements=None  Decoupling=off  VsMag0=0  VrMag0=0  VsAngle0=0  VrAngle0=0  IsMag0=0  IrMag0=0  IsAngle0=0  IrAngle0=0
      settings: SourceProductBaseCode=PS
  Line 48 : spsDistributedParametersLineLib/Distributed Parameters Line  Phases=3  Length=0.3  Frequency=50  Resistance=[0.80718830189013 0.0486237908083191 0.0486712220507153;0.0486237908083191 0.807093436079969 0.0486237934466192;0.0486712220507153 0.0486237934466192 0.80718830189013]  Inductance=[0.00279786707424938 0.00133270803418135 0.00132951476746136;0.00133270803418135 0.00279817608385787 0.00133799988507366;0.00132951476746136 0.00133799988507366 0.00279786707424938]  Capacitance=[7.73340098830622e-09 -1.79942827973291e-09 -1.73218055098733e-09;-1.79942827973291e-09 7.66505189233746e-09 -1.83375898618858e-09;-1.73218055098733e-09 -1.83375898618858e-09 7.749673531177e-09]  x1=[55.3555008057422 9831.4769944952 9831.45256680509;314.159265358979 314.159265358979 314.159265358979;1.07790763419893 -0.194668625001565 -1.76559166439652]  x2=[55.3555063663541 9831.47760181367 9831.45317514871;314.159265358979 314.159265358979 314.159265358979;1.07790758127811 -0.194668726500106 -1.7655917667403]  x3=[0.0482318691492677 24.9458576422003 25.1358615427219;314.159265358979 314.159265358979 314.159265358979;1.07745938290095 -0.195020166467593 -1.76594350325459]  x4=[0.0482318691604725 24.9458576424152 25.1358615428812;314.159265358979 314.159265358979 314.159265358979;1.07790758110099 -0.194668726500605 -1.76559176673969]  x5=1.42674452918375e-06  V1=ones(3,3)  V2=ones(3,3)  I1=ones(3,3)  I2=ones(3,3)  nHarmo=1  Measurements=None  Decoupling=off  VsMag0=0  VrMag0=0  VsAngle0=0  VrAngle0=0  IsMag0=0  IrMag0=0  IsAngle0=0  IrAngle0=0
      settings: SourceProductBaseCode=PS
  Line 49 : spsDistributedParametersLineLib/Distributed Parameters Line  Phases=3  Length=0.26  Frequency=50  Resistance=[0.646656091154803 0.0486237908083191 0.0486712220507153;0.0486237908083191 0.646561225344642 0.0486237934466192;0.0486712220507153 0.0486237934466192 0.646656091154803]  Inductance=[0.00282448912315926 0.00133270803418135 0.00132951476746136;0.00133270803418135 0.00282479813276775 0.00133799988507366;0.00132951476746136 0.00133799988507366 0.00282448912315926]  Capacitance=[7.89543174552926e-09 -1.85986777702161e-09 -1.7901190036642e-09;-1.85986777702161e-09 7.82540023894543e-09 -1.8957321828871e-09;-1.7901190036642e-09 -1.8957321828871e-09 7.91264394645417e-09]  x1=[132.042752270136 9831.39156427917 9831.28920891362;314.159265358979 314.159265358979 314.159265358979;1.01369806670442 -0.190316179557876 -1.76127884230239]  x2=[132.105723330459 9826.65273155558 9826.56698331564;314.159265358979 314.159265358979 314.159265358979;1.01374657267379 -0.190524082392513 -1.76148675247754]  x3=[0.211618922637013 6.68592407433364 6.5682555179452;314.159265358979 314.159265358979 314.159265358979;0.448020210141764 1.41239806602838 -0.183847755960689]  x4=[0.124854144417532 50.6704005813682 50.8673654780052;314.159265358979 314.159265358979 314.159265358979;2.15252957530103 -0.32284189823949 -1.89102198144784]  x5=1.2457829052789e-06  V1=ones(3,3)  V2=ones(3,3)  I1=ones(3,3)  I2=ones(3,3)  nHarmo=1  Measurements=None  Decoupling=off  VsMag0=0  VrMag0=0  VsAngle0=0  VrAngle0=0  IsMag0=0  IrMag0=0  IsAngle0=0  IrAngle0=0
      settings: SourceProductBaseCode=PS
  Line 5 : spsDistributedParametersLineLib/Distributed Parameters Line  Phases=3  Length=0.5  Frequency=50  Resistance=[0.646656091154803 0.0486237908083191 0.0486712220507153;0.0486237908083191 0.646561225344642 0.0486237934466192;0.0486712220507153 0.0486237934466192 0.646656091154803]  Inductance=[0.00282448912315926 0.00133270803418135 0.00132951476746136;0.00133270803418135 0.00282479813276775 0.00133799988507366;0.00132951476746136 0.00133799988507366 0.00282448912315926]  Capacitance=[7.89543174552926e-09 -1.85986777702161e-09 -1.7901190036642e-09;-1.85986777702161e-09 7.82540023894543e-09 -1.8957321828871e-09;-1.7901190036642e-09 -1.8957321828871e-09 7.91264394645417e-09]  x1=[131.754758180297 9848.08598665184 9847.5835251728;314.159265358979 314.159265358979 314.159265358979;1.0692001938948 2.25883211601059 -2.4533094733695]  x2=[131.763809776127 9846.88411593864 9846.39278960383;314.159265358979 314.159265358979 314.159265358979;1.06922206016094 2.25876099700567 -2.45337954210898]  x3=[0.12205695417996 21.4316560738869 21.6511868988184;314.159265358979 314.159265358979 314.159265358979;1.0061450726819 2.28205241582183 -2.43063563976]  x4=[0.108799290266388 28.671683601086 28.8337765425635;314.159265358979 314.159265358979 314.159265358979;1.13917542434306 2.24089133858056 -2.47091990390586]  x5=2.39573635630557e-06  V1=ones(3,3)  V2=ones(3,3)  I1=ones(3,3)  I2=ones(3,3)  nHarmo=1  Measurements=None  Decoupling=off  VsMag0=0  VrMag0=0  VsAngle0=0  VrAngle0=0  IsMag0=0  IrMag0=0  IsAngle0=0  IrAngle0=0
      settings: SourceProductBaseCode=PS
  Line 50 : spsDistributedParametersLineLib/Distributed Parameters Line  Phases=3  Length=0.02  Frequency=50  Resistance=[0.476003738225748 0.351747138225748 0.351747138225748;0.351747138225748 0.476003738225748 0.351747138225748;0.351747138225748 0.351747138225748 0.476003738225748]  Inductance=[0.000705954362986426 0.000459934243504405 0.000459934243504405;0.000459934243504405 0.000705954362986426 0.000459934243504405;0.000459934243504405 0.000459934243504405 0.000705954362986426]  Capacitance=[5.7561313269996e-07 -1.37543883484145e-07 -1.37543912800485e-07;-1.37543883484145e-07 5.75613027339387e-07 -1.37543875208088e-07;-1.37543912800485e-07 -1.37543875208088e-07 5.75613005057695e-07]  x1=[4.06087543990332 9838.61961804728 9839.35661781269;314.159265358979 314.159265358979 314.159265358979;1.25987815291883 -0.10817810706952 -1.67899323535444]  x2=[4.06113764319374 9838.54539143333 9839.28246477345;314.159265358979 314.159265358979 314.159265358979;1.25941141303888 -0.108180633306651 -1.67899579353961]  x3=[0.07989568254927 503.678799363723 503.681443480593;314.159265358979 314.159265358979 314.159265358979;0.14593271713554 -0.0959437944274121 -1.66696749990902]  x4=[0.10384893670745 555.711215935211 555.785404897829;314.159265358979 314.159265358979 314.159265358979;2.02153844805463 -0.119348585311048 -1.68997329609436]  x5=4.42086352438419e-07  V1=ones(3,3)  V2=ones(3,3)  I1=ones(3,3)  I2=ones(3,3)  nHarmo=1  Measurements=None  Decoupling=off  VsMag0=0  VrMag0=0  VsAngle0=0  VrAngle0=0  IsMag0=0  IrMag0=0  IsAngle0=0  IrAngle0=0
      settings: SourceProductBaseCode=PS
  Line 51 : spsDistributedParametersLineLib/Distributed Parameters Line  Phases=3  Length=1.7101  Frequency=50  Resistance=[0.646656091154803 0.0486237908083191 0.0486712220507153;0.0486237908083191 0.646561225344642 0.0486237934466192;0.0486712220507153 0.0486237934466192 0.646656091154803]  Inductance=[0.00282448912315926 0.00133270803418135 0.00132951476746136;0.00133270803418135 0.00282479813276775 0.00133799988507366;0.00132951476746136 0.00133799988507366 0.00282448912315926]  Capacitance=[7.89543174552926e-09 -1.85986777702161e-09 -1.7901190036642e-09;-1.85986777702161e-09 7.82540023894543e-09 -1.8957321828871e-09;-1.7901190036642e-09 -1.8957321828871e-09 7.91264394645417e-09]  x1=[131.560969710531 9869.14674526761 9868.91738624598;314.159265358979 314.159265358979 314.159265358979;1.0113175454731 -0.190307546709514 -1.76127165790901]  x2=[131.978388759833 9837.58324201183 9837.46109872544;314.159265358979 314.159265358979 314.159265358979;1.01169767234449 -0.191790767382132 -1.7627546107336]  x3=[0.213451463453635 6.21731681945902 6.07979797020263;314.159265358979 314.159265358979 314.159265358979;0.451044106992652 1.52944552629848 -0.0662872569640212]  x4=[0.123495827937136 51.3564310859456 51.5543155604359;314.159265358979 314.159265358979 314.159265358979;2.17046626182479 -0.312048404503478 -1.88030043645935]  x5=8.19389748583632e-06  V1=ones(3,3)  V2=ones(3,3)  I1=ones(3,3)  I2=ones(3,3)  nHarmo=1  Measurements=None  Decoupling=off  VsMag0=0  VrMag0=0  VsAngle0=0  VrAngle0=0  IsMag0=0  IrMag0=0  IsAngle0=0  IrAngle0=0
      settings: SourceProductBaseCode=PS
  Line 52 : spsDistributedParametersLineLib/Distributed Parameters Line  Phases=3  Length=0.02  Frequency=50  Resistance=[0.646656091154803 0.0486237908083191 0.0486712220507153;0.0486237908083191 0.646561225344642 0.0486237934466192;0.0486712220507153 0.0486237934466192 0.646656091154803]  Inductance=[0.00282448912315926 0.00133270803418135 0.00132951476746136;0.00133270803418135 0.00282479813276775 0.00133799988507366;0.00132951476746136 0.00133799988507366 0.00282448912315926]  Capacitance=[7.89543174552926e-09 -1.85986777702161e-09 -1.7901190036642e-09;-1.85986777702161e-09 7.82540023894543e-09 -1.8957321828871e-09;-1.7901190036642e-09 -1.8957321828871e-09 7.91264394645417e-09]  x1=[131.560969710531 9869.14674526761 9868.91738624598;314.159265358979 314.159265358979 314.159265358979;1.01386162857673 -0.188286439773996 -1.7592486270228]  x2=[131.561045863184 9869.13510874332 9868.9057672105;314.159265358979 314.159265358979 314.159265358979;1.01386197461704 -0.188286842544668 -1.75924902541665]  x3=[0.11695446421553 24.3537247091606 24.5458082735576;314.159265358979 314.159265358979 314.159265358979;1.00201249115567 -0.177322213898108 -1.74837735145565]  x4=[0.113116730285478 25.8797370451913 26.0722429168796;314.159265358979 314.159265358979 314.159265358979;1.02608252882494 -0.198627733492271 -1.76950703199435]  x5=9.5829454252223e-08  V1=ones(3,3)  V2=ones(3,3)  I1=ones(3,3)  I2=ones(3,3)  nHarmo=1  Measurements=None  Decoupling=off  VsMag0=0  VrMag0=0  VsAngle0=0  VrAngle0=0  IsMag0=0  IrMag0=0  IsAngle0=0  IrAngle0=0
      settings: SourceProductBaseCode=PS
  Line 53 : spsDistributedParametersLineLib/Distributed Parameters Line  Phases=3  Length=0.02  Frequency=50  Resistance=[0.646656091154803 0.0486237908083191 0.0486712220507153;0.0486237908083191 0.646561225344642 0.0486237934466192;0.0486712220507153 0.0486237934466192 0.646656091154803]  Inductance=[0.00282448912315926 0.00133270803418135 0.00132951476746136;0.00133270803418135 0.00282479813276775 0.00133799988507366;0.00132951476746136 0.00133799988507366 0.00282448912315926]  Capacitance=[7.89543174552926e-09 -1.85986777702161e-09 -1.7901190036642e-09;-1.85986777702161e-09 7.82540023894543e-09 -1.8957321828871e-09;-1.7901190036642e-09 -1.8957321828871e-09 7.91264394645417e-09]  x1=[131.556006639317 9869.52740554651 9869.296774612;314.159265358979 314.159265358979 314.159265358979;1.01385683970015 -0.188268714759086 -1.75923090904831]  x2=[131.560969710531 9869.14674526761 9868.91738624598;314.159265358979 314.159265358979 314.159265358979;1.01386162857673 -0.188286439773996 -1.7592486270228]  x3=[0.215955858122158 6.63674141741294 6.48338169673315;314.159265358979 314.159265358979 314.159265358979;0.452925789233531 1.63684766234951 0.0450227492992415]  x4=[0.124193776578071 52.2974202298391 52.4965439023838;314.159265358979 314.159265358979 314.159265358979;2.19491193213471 -0.311421668078114 -1.87969294392368]  x5=9.5829454252223e-08  V1=ones(3,3)  V2=ones(3,3)  I1=ones(3,3)  I2=ones(3,3)  nHarmo=1  Measurements=None  Decoupling=off  VsMag0=0  VrMag0=0  VsAngle0=0  VrAngle0=0  IsMag0=0  IrMag0=0  IsAngle0=0  IrAngle0=0
      settings: SourceProductBaseCode=PS
  Line 54 : spsDistributedParametersLineLib/Distributed Parameters Line  Phases=3  Length=1.15  Frequency=50  Resistance=[0.646656091154803 0.0486237908083191 0.0486712220507153;0.0486237908083191 0.646561225344642 0.0486237934466192;0.0486712220507153 0.0486237934466192 0.646656091154803]  Inductance=[0.00282448912315926 0.00133270803418135 0.00132951476746136;0.00133270803418135 0.00282479813276775 0.00133799988507366;0.00132951476746136 0.00133799988507366 0.00282448912315926]  Capacitance=[7.89543174552926e-09 -1.85986777702161e-09 -1.7901190036642e-09;-1.85986777702161e-09 7.82540023894543e-09 -1.8957321828871e-09;-1.7901190036642e-09 -1.8957321828871e-09 7.91264394645417e-09]  x1=[131.556006639317 9869.52740554651 9869.296774612;314.159265358979 314.159265358979 314.159265358979;1.0121558670316 -0.189620025827742 -1.76058350646941]  x2=[131.563010144033 9868.60064496095 9868.37156927628;314.159265358979 314.159265358979 314.159265358979;1.01218117676731 -0.189655701613067 -1.76061886165816]  x3=[0.11768889584068 24.0050111880476 24.1965041516975;314.159265358979 314.159265358979 314.159265358979;0.991169334611457 -0.176255603993913 -1.74736277963593]  x4=[0.112285431951849 26.1650557507942 26.3571322920126;314.159265358979 314.159265358979 314.159265358979;1.03240532413202 -0.203234327046454 -1.77407500070752]  x5=5.51019361950282e-06  V1=ones(3,3)  V2=ones(3,3)  I1=ones(3,3)  I2=ones(3,3)  nHarmo=1  Measurements=None  Decoupling=off  VsMag0=0  VrMag0=0  VsAngle0=0  VrAngle0=0  IsMag0=0  IrMag0=0  IsAngle0=0  IrAngle0=0
      settings: SourceProductBaseCode=PS
  Line 55 : spsDistributedParametersLineLib/Distributed Parameters Line  Phases=3  Length=0.18999  Frequency=50  Resistance=[0.646656091154803 0.0486237908083191 0.0486712220507153;0.0486237908083191 0.646561225344642 0.0486237934466192;0.0486712220507153 0.0486237934466192 0.646656091154803]  Inductance=[0.00282448912315926 0.00133270803418135 0.00132951476746136;0.00133270803418135 0.00282479813276775 0.00133799988507366;0.00132951476746136 0.00133799988507366 0.00282448912315926]  Capacitance=[7.89543174552926e-09 -1.85986777702161e-09 -1.7901190036642e-09;-1.85986777702161e-09 7.82540023894543e-09 -1.8957321828871e-09;-1.7901190036642e-09 -1.8957321828871e-09 7.91264394645417e-09]  x1=[131.563010144033 9868.60064496095 9868.37156927628;314.159265358979 314.159265358979 314.159265358979;1.01362626594565 -0.188507673171456 -1.75946974037477]  x2=[131.563338462186 9868.55483473402 9868.3258702577;314.159265358979 314.159265358979 314.159265358979;1.01362684394256 -0.188507834436501 -1.75946988818402]  x3=[0.115583096583862 24.8536771339215 25.0457956601435;314.159265358979 314.159265358979 314.159265358979;1.00689332327359 -0.181088149680304 -1.7521106763789]  x4=[0.114461236858345 25.3657250116119 25.5580411394045;314.159265358979 314.159265358979 314.159265358979;1.02013838190988 -0.196002501212929 -1.76690660772535]  x5=9.10331900668992e-07  V1=ones(3,3)  V2=ones(3,3)  I1=ones(3,3)  I2=ones(3,3)  nHarmo=1  Measurements=None  Decoupling=off  VsMag0=0  VrMag0=0  VsAngle0=0  VrAngle0=0  IsMag0=0  IrMag0=0  IsAngle0=0  IrAngle0=0
      settings: SourceProductBaseCode=PS
  Line 56 : spsDistributedParametersLineLib/Distributed Parameters Line  Phases=3  Length=0.34003  Frequency=50  Resistance=[0.646656091154803 0.0486237908083191 0.0486712220507153;0.0486237908083191 0.646561225344642 0.0486237934466192;0.0486712220507153 0.0486237934466192 0.646656091154803]  Inductance=[0.00282448912315926 0.00133270803418135 0.00132951476746136;0.00133270803418135 0.00282479813276775 0.00133799988507366;0.00132951476746136 0.00133799988507366 0.00282448912315926]  Capacitance=[7.89543174552926e-09 -1.85986777702161e-09 -1.7901190036642e-09;-1.85986777702161e-09 7.82540023894543e-09 -1.8957321828871e-09;-1.7901190036642e-09 -1.8957321828871e-09 7.91264394645417e-09]  x1=[131.563010144033 9868.60064496095 9868.37156927628;314.159265358979 314.159265358979 314.159265358979;1.01340041290213 -0.188687098580961 -1.75964933658456]  x2=[131.564408197594 9868.40458095763 9868.1757584693;314.159265358979 314.159265358979 314.159265358979;1.01340714061792 -0.188696839995956 -1.75965900287874]  x3=[0.117163659160691 24.2796662386408 24.4716122223081;314.159265358979 314.159265358979 314.159265358979;1.00065593876547 -0.181639420607069 -1.75267859029351]  x4=[0.112878396681563 25.9305987897049 26.1229494775985;314.159265358979 314.159265358979 314.159265358979;1.02611400717747 -0.19568922502469 -1.76658298646914]  x5=1.62924446646917e-06  V1=ones(3,3)  V2=ones(3,3)  I1=ones(3,3)  I2=ones(3,3)  nHarmo=1  Measurements=None  Decoupling=off  VsMag0=0  VrMag0=0  VsAngle0=0  VrAngle0=0  IsMag0=0  IrMag0=0  IsAngle0=0  IrAngle0=0
      settings: SourceProductBaseCode=PS
  Line 57 : spsDistributedParametersLineLib/Distributed Parameters Line  Phases=3  Length=0.12001  Frequency=50  Resistance=[0.646656091154803 0.0486237908083191 0.0486712220507153;0.0486237908083191 0.646561225344642 0.0486237934466192;0.0486712220507153 0.0486237934466192 0.646656091154803]  Inductance=[0.00282448912315926 0.00133270803418135 0.00132951476746136;0.00133270803418135 0.00282479813276775 0.00133799988507366;0.00132951476746136 0.00133799988507366 0.00282448912315926]  Capacitance=[7.89543174552926e-09 -1.85986777702161e-09 -1.7901190036642e-09;-1.85986777702161e-09 7.82540023894543e-09 -1.8957321828871e-09;-1.7901190036642e-09 -1.8957321828871e-09 7.91264394645417e-09]  x1=[131.564408197594 9868.40458095763 9868.1757584693;314.159265358979 314.159265358979 314.159265358979;1.01373833354405 -0.188433728968234 -1.75939564138795]  x2=[131.564650090993 9868.36705005654 9868.13827229414;314.159265358979 314.159265358979 314.159265358979;1.01373966943552 -0.188435465973585 -1.75939736330211]  x3=[0.116169608082311 24.6714190521824 24.8635595488729;314.159265358979 314.159265358979 314.159265358979;1.00781412638493 -0.184192137028728 -1.75519234581304]  x4=[0.113883880502427 25.5500715661833 25.7424274724326;314.159265358979 314.159265358979 314.159265358979;1.01960032862429 -0.192672213996611 -1.7635983295754]  x5=5.75024640240464e-07  V1=ones(3,3)  V2=ones(3,3)  I1=ones(3,3)  I2=ones(3,3)  nHarmo=1  Measurements=None  Decoupling=off  VsMag0=0  VrMag0=0  VsAngle0=0  VrAngle0=0  IsMag0=0  IrMag0=0  IsAngle0=0  IrAngle0=0
      settings: SourceProductBaseCode=PS
  Line 58 : spsDistributedParametersLineLib/Distributed Parameters Line  Phases=3  Length=0.82  Frequency=50  Resistance=[0.646656091154803 0.0486237908083191 0.0486712220507153;0.0486237908083191 0.646561225344642 0.0486237934466192;0.0486712220507153 0.0486237934466192 0.646656091154803]  Inductance=[0.00282448912315926 0.00133270803418135 0.00132951476746136;0.00133270803418135 0.00282479813276775 0.00133799988507366;0.00132951476746136 0.00133799988507366 0.00282448912315926]  Capacitance=[7.89543174552926e-09 -1.85986777702161e-09 -1.7901190036642e-09;-1.85986777702161e-09 7.82540023894543e-09 -1.8957321828871e-09;-1.7901190036642e-09 -1.8957321828871e-09 7.91264394645417e-09]  x1=[131.564408197594 9868.40458095763 9868.1757584693;314.159265358979 314.159265358979 314.159265358979;1.01268464871374 -0.189270812361993 -1.76023352162583]  x2=[131.565970434362 9868.18079763976 9867.95226618196;314.159265358979 314.159265358979 314.159265358979;1.01269225766996 -0.189281481605769 -1.76024410474037]  x3=[0.115987880728862 24.7043745423781 24.8962233397174;314.159265358979 314.159265358979 314.159265358979;1.00625275791035 -0.186167754005847 -1.75716661090434]  x4=[0.113988385613898 25.4764154316575 25.6684508052301;314.159265358979 314.159265358979 314.159265358979;1.01799171389719 -0.193256382765175 -1.76418565879477]  x5=3.92900762434114e-06  V1=ones(3,3)  V2=ones(3,3)  I1=ones(3,3)  I2=ones(3,3)  nHarmo=1  Measurements=None  Decoupling=off  VsMag0=0  VrMag0=0  VsAngle0=0  VrAngle0=0  IsMag0=0  IrMag0=0  IsAngle0=0  IrAngle0=0
      settings: SourceProductBaseCode=PS
  Line 59 : spsDistributedParametersLineLib/Distributed Parameters Line  Phases=3  Length=1.11  Frequency=50  Resistance=[0.646656091154803 0.0486237908083191 0.0486712220507153;0.0486237908083191 0.646561225344642 0.0486237934466192;0.0486712220507153 0.0486237934466192 0.646656091154803]  Inductance=[0.00282448912315926 0.00133270803418135 0.00132951476746136;0.00133270803418135 0.00282479813276775 0.00133799988507366;0.00132951476746136 0.00133799988507366 0.00282448912315926]  Capacitance=[7.89543174552926e-09 -1.85986777702161e-09 -1.7901190036642e-09;-1.85986777702161e-09 7.82540023894543e-09 -1.8957321828871e-09;-1.7901190036642e-09 -1.8957321828871e-09 7.91264394645417e-09]  x1=[131.273424847613 9891.535924883 9891.23316090554;314.159265358979 314.159265358979 314.159265358979;1.01192646910363 -0.188554027050442 -1.75951813380569]  x2=[131.556006639317 9869.52740554651 9869.296774612;314.159265358979 314.159265358979 314.159265358979;1.0122160784535 -0.189572191807612 -1.76053562691468]  x3=[0.21937805723341 7.25378835382827 7.08320044760709;314.159265358979 314.159265358979 314.159265358979;0.446790589283102 1.76320055701698 0.176174840366232]  x4=[0.125448343337879 53.3572202530781 53.5553860501431;314.159265358979 314.159265358979 314.159265358979;2.22087925775378 -0.316205500251278 -1.88450305404549]  x5=5.31853471099837e-06  V1=ones(3,3)  V2=ones(3,3)  I1=ones(3,3)  I2=ones(3,3)  nHarmo=1  Measurements=None  Decoupling=off  VsMag0=0  VrMag0=0  VsAngle0=0  VrAngle0=0  IsMag0=0  IrMag0=0  IsAngle0=0  IrAngle0=0
      settings: SourceProductBaseCode=PS
  Line 6 : spsDistributedParametersLineLib/Distributed Parameters Line  Phases=3  Length=0.23  Frequency=50  Resistance=[0.646656091154803 0.0486237908083191 0.0486712220507153;0.0486237908083191 0.646561225344642 0.0486237934466192;0.0486712220507153 0.0486237934466192 0.646656091154803]  Inductance=[0.00282448912315926 0.00133270803418135 0.00132951476746136;0.00133270803418135 0.00282479813276775 0.00133799988507366;0.00132951476746136 0.00133799988507366 0.00282448912315926]  Capacitance=[7.89543174552926e-09 -1.85986777702161e-09 -1.7901190036642e-09;-1.85986777702161e-09 7.82540023894543e-09 -1.8957321828871e-09;-1.7901190036642e-09 -1.8957321828871e-09 7.91264394645417e-09]  x1=[131.749735782929 9848.86865393328 9848.36073374528;314.159265358979 314.159265358979 314.159265358979;1.06958501865401 2.25919512382356 -2.45294673850185]  x2=[131.754758180297 9848.08598665184 9847.5835251728;314.159265358979 314.159265358979 314.159265358979;1.06960662099259 2.25915499564647 -2.45298628637507]  x3=[0.126112838961531 20.1680233582042 20.3872694855582;314.159265358979 314.159265358979 314.159265358979;1.00531074945902 2.30806580941596 -2.40491406161109]  x4=[0.104823513316601 29.9859395813574 30.1480421043991;314.159265358979 314.159265358979 314.159265358979;1.14657930023752 2.22606918905994 -2.48568534590631]  x5=1.10203872390056e-06  V1=ones(3,3)  V2=ones(3,3)  I1=ones(3,3)  I2=ones(3,3)  nHarmo=1  Measurements=None  Decoupling=off  VsMag0=0  VrMag0=0  VsAngle0=0  VrAngle0=0  IsMag0=0  IrMag0=0  IsAngle0=0  IrAngle0=0
      settings: SourceProductBaseCode=PS
  Line 60 : spsDistributedParametersLineLib/Distributed Parameters Line  Phases=3  Length=0.20999  Frequency=50  Resistance=[0.646656091154803 0.0486237908083191 0.0486712220507153;0.0486237908083191 0.646561225344642 0.0486237934466192;0.0486712220507153 0.0486237934466192 0.646656091154803]  Inductance=[0.00282448912315926 0.00133270803418135 0.00132951476746136;0.00133270803418135 0.00282479813276775 0.00133799988507366;0.00132951476746136 0.00133799988507366 0.00282448912315926]  Capacitance=[7.89543174552926e-09 -1.85986777702161e-09 -1.7901190036642e-09;-1.85986777702161e-09 7.82540023894543e-09 -1.8957321828871e-09;-1.7901190036642e-09 -1.8957321828871e-09 7.91264394645417e-09]  x1=[131.273424847613 9891.535924883 9891.23316090554;314.159265358979 314.159265358979 314.159265358979;1.01328124114913 -0.187477749639025 -1.75844083185439]  x2=[131.321087888507 9888.25512471752 9887.96648693994;314.159265358979 314.159265358979 314.159265358979;1.01332528979424 -0.187666074827015 -1.75862890768003]  x3=[0.205289199924438 3.96176633180301 3.963931265872;314.159265358979 314.159265358979 314.159265358979;0.474357508025624 0.908943294288709 -0.719007950951876]  x4=[0.118080358493603 48.6443096903409 48.8222260733637;314.159265358979 314.159265358979 314.159265358979;2.11499594246175 -0.260219622182137 -1.82872313133347]  x5=1.00616135492121e-06  V1=ones(3,3)  V2=ones(3,3)  I1=ones(3,3)  I2=ones(3,3)  nHarmo=1  Measurements=None  Decoupling=off  VsMag0=0  VrMag0=0  VsAngle0=0  VrAngle0=0  IsMag0=0  IrMag0=0  IsAngle0=0  IrAngle0=0
      settings: SourceProductBaseCode=PS
  Line 61 : spsDistributedParametersLineLib/Distributed Parameters Line  Phases=3  Length=0.23002  Frequency=50  Resistance=[0.476003738225748 0.351747138225748 0.351747138225748;0.351747138225748 0.476003738225748 0.351747138225748;0.351747138225748 0.351747138225748 0.476003738225748]  Inductance=[0.000705954362986426 0.000459934243504405 0.000459934243504405;0.000459934243504405 0.000705954362986426 0.000459934243504405;0.000459934243504405 0.000459934243504405 0.000705954362986426]  Capacitance=[5.7561313269996e-07 -1.37543883484145e-07 -1.37543912800485e-07;-1.37543883484145e-07 5.75613027339387e-07 -1.37543875208088e-07;-1.37543912800485e-07 -1.37543875208088e-07 5.75613005057695e-07]  x1=[2.69067392863843 9889.29674491797 9889.87525179247;314.159265358979 314.159265358979 314.159265358979;1.24161148608124 -0.106722370837188 -1.67753578044334]  x2=[2.69445799483125 9888.56218635767 9889.14229167894;314.159265358979 314.159265358979 314.159265358979;1.23335469315781 -0.106753432792825 -1.67756714768376]  x3=[0.0760845460472585 508.507678130699 508.530725631183;314.159265358979 314.159265358979 314.159265358979;-0.0893585933812519 -0.0997995373660825 -1.67081312171309]  x4=[0.0918009215456045 555.136410682875 555.174164015881;314.159265358979 314.159265358979 314.159265358979;2.17083752003826 -0.11401079960911 -1.68464099139257]  x5=5.08443513939426e-06  V1=ones(3,3)  V2=ones(3,3)  I1=ones(3,3)  I2=ones(3,3)  nHarmo=1  Measurements=None  Decoupling=off  VsMag0=0  VrMag0=0  VsAngle0=0  VrAngle0=0  IsMag0=0  IrMag0=0  IsAngle0=0  IrAngle0=0
      settings: SourceProductBaseCode=PS
  Line 62 : spsDistributedParametersLineLib/Distributed Parameters Line  Phases=3  Length=0.24001  Frequency=50  Resistance=[0.646656091154803 0.0486237908083191 0.0486712220507153;0.0486237908083191 0.646561225344642 0.0486237934466192;0.0486712220507153 0.0486237934466192 0.646656091154803]  Inductance=[0.00282448912315926 0.00133270803418135 0.00132951476746136;0.00133270803418135 0.00282479813276775 0.00133799988507366;0.00132951476746136 0.00133799988507366 0.00282448912315926]  Capacitance=[7.89543174552926e-09 -1.85986777702161e-09 -1.7901190036642e-09;-1.85986777702161e-09 7.82540023894543e-09 -1.8957321828871e-09;-1.7901190036642e-09 -1.8957321828871e-09 7.91264394645417e-09]  x1=[131.15149650027 9900.04928765204 9899.71179690672;314.159265358979 314.159265358979 314.159265358979;1.01319873064665 -0.187079277015596 -1.7580420298444]  x2=[131.273424847562 9891.53592488655 9891.23316090909;314.159265358979 314.159265358979 314.159265358979;1.01323605247693 -0.187513649070953 -1.75847676546003]  x3=[0.337008529917423 27.9974318631287 27.7484919882165;314.159265358979 314.159265358979 314.159265358979;0.201460729802306 2.57725918359549 1.01310682389371]  x4=[0.244470286416648 77.0778180346214 77.263099526498;314.159265358979 314.159265358979 314.159265358979;2.5943105950515 -0.321524423337029 -1.88867043536489]  x5=1.1500013657538e-06  V1=ones(3,3)  V2=ones(3,3)  I1=ones(3,3)  I2=ones(3,3)  nHarmo=1  Measurements=None  Decoupling=off  VsMag0=0  VrMag0=0  VsAngle0=0  VrAngle0=0  IsMag0=0  IrMag0=0  IsAngle0=0  IrAngle0=0
      settings: SourceProductBaseCode=PS
  Line 63 : spsDistributedParametersLineLib/Distributed Parameters Line  Phases=3  Length=0.02  Frequency=50  Resistance=[0.646656091154803 0.0486237908083191 0.0486712220507153;0.0486237908083191 0.646561225344642 0.0486237934466192;0.0486712220507153 0.0486237934466192 0.646656091154803]  Inductance=[0.00282448912315926 0.00133270803418135 0.00132951476746136;0.00133270803418135 0.00282479813276775 0.00133799988507366;0.00132951476746136 0.00133799988507366 0.00282448912315926]  Capacitance=[7.89543174552926e-09 -1.85986777702161e-09 -1.7901190036642e-09;-1.85986777702161e-09 7.82540023894543e-09 -1.8957321828871e-09;-1.7901190036642e-09 -1.8957321828871e-09 7.91264394645417e-09]  x1=[131.15149650027 9900.04928765204 9899.71179690672;314.159265358979 314.159265358979 314.159265358979;1.01352990851993 -0.186816177946379 -1.7577786803235]  x2=[131.151537794759 9900.0432680569 9899.70579003085;314.159265358979 314.159265358979 314.159265358979;1.01353002118718 -0.186816259237808 -1.75777875967023]  x3=[0.115470330715768 24.8509063907571 25.0434189301217;314.159265358979 314.159265358979 314.159265358979;1.00610895259527 -0.178660372050177 -1.74968834416178]  x4=[0.113874527395509 25.5386411495266 25.7313834073222;314.159265358979 314.159265358979 314.159265358979;1.02102465769206 -0.194776025299464 -1.76567640371142]  x5=9.5829454252223e-08  V1=ones(3,3)  V2=ones(3,3)  I1=ones(3,3)  I2=ones(3,3)  nHarmo=1  Measurements=None  Decoupling=off  VsMag0=0  VrMag0=0  VsAngle0=0  VrAngle0=0  IsMag0=0  IrMag0=0  IsAngle0=0  IrAngle0=0
      settings: SourceProductBaseCode=PS
  Line 64 : spsDistributedParametersLineLib/Distributed Parameters Line  Phases=3  Length=0.5  Frequency=50  Resistance=[0.646656091154803 0.0486237908083191 0.0486712220507153;0.0486237908083191 0.646561225344642 0.0486237934466192;0.0486712220507153 0.0486237934466192 0.646656091154803]  Inductance=[0.00282448912315926 0.00133270803418135 0.00132951476746136;0.00133270803418135 0.00282479813276775 0.00133799988507366;0.00132951476746136 0.00133799988507366 0.00282448912315926]  Capacitance=[7.89543174552926e-09 -1.85986777702161e-09 -1.7901190036642e-09;-1.85986777702161e-09 7.82540023894543e-09 -1.8957321828871e-09;-1.7901190036642e-09 -1.8957321828871e-09 7.91264394645417e-09]  x1=[130.896401502654 9917.93852384676 9917.52837515293;314.159265358979 314.159265358979 314.159265358979;1.01272676072288 -0.186485317185372 -1.75744764649431]  x2=[131.15149650027 9900.04928765204 9899.71179690672;314.159265358979 314.159265358979 314.159265358979;1.01280737145718 -0.187390186187932 -1.75835323498025]  x3=[0.338063259702629 28.3491130111897 28.0995909214384;314.159265358979 314.159265358979 314.159265358979;0.200354052669773 2.57395781975361 1.00969221841147]  x4=[0.245354556312368 77.4470667624491 77.6318066428181;314.159265358979 314.159265358979 314.159265358979;2.59758723245899 -0.323567314163692 -1.89072525588915]  x5=2.39573635630557e-06  V1=ones(3,3)  V2=ones(3,3)  I1=ones(3,3)  I2=ones(3,3)  nHarmo=1  Measurements=None  Decoupling=off  VsMag0=0  VrMag0=0  VsAngle0=0  VrAngle0=0  IsMag0=0  IrMag0=0  IsAngle0=0  IrAngle0=0
      settings: SourceProductBaseCode=PS
  Line 65 : spsDistributedParametersLineLib/Distributed Parameters Line  Phases=3  Length=0.23  Frequency=50  Resistance=[0.646656091154803 0.0486237908083191 0.0486712220507153;0.0486237908083191 0.646561225344642 0.0486237934466192;0.0486712220507153 0.0486237934466192 0.646656091154803]  Inductance=[0.00282448912315926 0.00133270803418135 0.00132951476746136;0.00133270803418135 0.00282479813276775 0.00133799988507366;0.00132951476746136 0.00133799988507366 0.00282448912315926]  Capacitance=[7.89543174552926e-09 -1.85986777702161e-09 -1.7901190036642e-09;-1.85986777702161e-09 7.82540023894543e-09 -1.8957321828871e-09;-1.7901190036642e-09 -1.8957321828871e-09 7.91264394645417e-09]  x1=[130.776470898154 9926.56913852249 9926.12505116031;314.159265358979 314.159265358979 314.159265358979;1.01308236260569 -0.185730239738517 -1.75669208327806]  x2=[130.896401502654 9917.93852384676 9917.52837515294;314.159265358979 314.159265358979 314.159265358979;1.01313318782067 -0.186162437549499 -1.75712445949988]  x3=[0.345072018942222 30.7988938346752 30.5511753409241;314.159265358979 314.159265358979 314.159265358979;0.205855984260785 2.58290676019646 1.01819775009686]  x4=[0.249431325120644 79.9643512032649 80.1488292932599;314.159265358979 314.159265358979 314.159265358979;2.62339801138026 -0.326760249454387 -1.89401608788156]  x5=1.10203872390056e-06  V1=ones(3,3)  V2=ones(3,3)  I1=ones(3,3)  I2=ones(3,3)  nHarmo=1  Measurements=None  Decoupling=off  VsMag0=0  VrMag0=0  VsAngle0=0  VrAngle0=0  IsMag0=0  IrMag0=0  IsAngle0=0  IrAngle0=0
      settings: SourceProductBaseCode=PS
  Line 66 : spsDistributedParametersLineLib/Distributed Parameters Line  Phases=3  Length=1.62  Frequency=50  Resistance=[0.80718830189013 0.0486237908083191 0.0486712220507153;0.0486237908083191 0.807093436079969 0.0486237934466192;0.0486712220507153 0.0486237934466192 0.80718830189013]  Inductance=[0.00279786707424938 0.00133270803418135 0.00132951476746136;0.00133270803418135 0.00279817608385787 0.00133799988507366;0.00132951476746136 0.00133799988507366 0.00279786707424938]  Capacitance=[7.73340098830622e-09 -1.79942827973291e-09 -1.73218055098733e-09;-1.79942827973291e-09 7.66505189233746e-09 -1.83375898618858e-09;-1.73218055098733e-09 -1.83375898618858e-09 7.749673531177e-09]  x1=[53.3104012264039 9926.65509988325 9926.28243860362;314.159265358979 314.159265358979 314.159265358979;1.07080536334471 -0.191665293218079 -1.76258875082596]  x2=[53.3107675967131 9926.65648549892 9926.28388669192;314.159265358979 314.159265358979 314.159265358979;1.0708047980231 -0.191668116755943 -1.7625915947463]  x3=[0.0464599290184069 25.1301446212904 25.3203715372516;314.159265358979 314.159265358979 314.159265358979;1.06727870369421 -0.193296723424129 -1.76422385403076]  x4=[0.0463682408066111 25.1487041416633 25.3389363044987;314.159265358979 314.159265358979 314.159265358979;1.07191485024146 -0.19193671829372 -1.76285813769938]  x5=7.70442045759223e-06  V1=ones(3,3)  V2=ones(3,3)  I1=ones(3,3)  I2=ones(3,3)  nHarmo=1  Measurements=None  Decoupling=off  VsMag0=0  VrMag0=0  VsAngle0=0  VrAngle0=0  IsMag0=0  IrMag0=0  IsAngle0=0  IrAngle0=0
      settings: SourceProductBaseCode=PS
  Line 67 : spsDistributedParametersLineLib/Distributed Parameters Line  Phases=3  Length=0.54002  Frequency=50  Resistance=[0.646656091154803 0.0486237908083191 0.0486712220507153;0.0486237908083191 0.646561225344642 0.0486237934466192;0.0486712220507153 0.0486237934466192 0.646656091154803]  Inductance=[0.00282448912315926 0.00133270803418135 0.00132951476746136;0.00133270803418135 0.00282479813276775 0.00133799988507366;0.00132951476746136 0.00133799988507366 0.00282448912315926]  Capacitance=[7.89543174552926e-09 -1.85986777702161e-09 -1.7901190036642e-09;-1.85986777702161e-09 7.82540023894543e-09 -1.8957321828871e-09;-1.7901190036642e-09 -1.8957321828871e-09 7.91264394645417e-09]  x1=[130.494546105913 9946.82998998348 9946.30618573429;314.159265358979 314.159265358979 314.159265358979;1.01249692339735 -0.18508721382624 -1.75604896658942]  x2=[130.776470898154 9926.56913852249 9926.12505116031;314.159265358979 314.159265358979 314.159265358979;1.01261569398029 -0.18610097731153 -1.75706317376699]  x3=[0.345164537322001 30.7435314803863 30.4956580105405;314.159265358979 314.159265358979 314.159265358979;0.204116790594438 2.58303183225723 1.01834494276494]  x4=[0.249734116896454 79.9652457323251 80.1497312095374;314.159265358979 314.159265358979 314.159265358979;2.62341355576043 -0.326352127048185 -1.89360416267025]  x5=2.58749109426427e-06  V1=ones(3,3)  V2=ones(3,3)  I1=ones(3,3)  I2=ones(3,3)  nHarmo=1  Measurements=None  Decoupling=off  VsMag0=0  VrMag0=0  VsAngle0=0  VrAngle0=0  IsMag0=0  IrMag0=0  IsAngle0=0  IrAngle0=0
      settings: SourceProductBaseCode=PS
  Line 68 : spsDistributedParametersLineLib/Distributed Parameters Line  Phases=3  Length=0.13998  Frequency=50  Resistance=[0.646656091154803 0.0486237908083191 0.0486712220507153;0.0486237908083191 0.646561225344642 0.0486237934466192;0.0486712220507153 0.0486237934466192 0.646656091154803]  Inductance=[0.00282448912315926 0.00133270803418135 0.00132951476746136;0.00133270803418135 0.00282479813276775 0.00133799988507366;0.00132951476746136 0.00133799988507366 0.00282448912315926]  Capacitance=[7.89543174552926e-09 -1.85986777702161e-09 -1.7901190036642e-09;-1.85986777702161e-09 7.82540023894543e-09 -1.8957321828871e-09;-1.7901190036642e-09 -1.8957321828871e-09 7.91264394645417e-09]  x1=[130.494546105913 9946.82998998348 9946.30618573429;314.159265358979 314.159265358979 314.159265358979;1.01309909782773 -0.184608825790926 -1.75557012316257]  x2=[130.49530648087 9946.71305313154 9946.18941024581;314.159265358979 314.159265358979 314.159265358979;1.01310295852149 -0.184613493237634 -1.75557474548442]  x3=[0.117013645843791 24.1787348195121 24.3714685571204;314.159265358979 314.159265358979 314.159265358979;0.996757089814386 -0.170803086287499 -1.74188624629639]  x4=[0.111195019439981 26.4445285054675 26.6377875429643;314.159265358979 314.159265358979 314.159265358979;1.03008406706403 -0.197396308553645 -1.76825458431165]  x5=6.70710350311308e-07  V1=ones(3,3)  V2=ones(3,3)  I1=ones(3,3)  I2=ones(3,3)  nHarmo=1  Measurements=None  Decoupling=off  VsMag0=0  VrMag0=0  VsAngle0=0  VrAngle0=0  IsMag0=0  IrMag0=0  IsAngle0=0  IrAngle0=0
      settings: SourceProductBaseCode=PS
  Line 69 : spsDistributedParametersLineLib/Distributed Parameters Line  Phases=3  Length=0.14997  Frequency=50  Resistance=[0.476003738225748 0.351747138225748 0.351747138225748;0.351747138225748 0.476003738225748 0.351747138225748;0.351747138225748 0.351747138225748 0.476003738225748]  Inductance=[0.000705954362986426 0.000459934243504405 0.000459934243504405;0.000459934243504405 0.000705954362986426 0.000459934243504405;0.000459934243504405 0.000459934243504405 0.000705954362986426]  Capacitance=[5.7561313269996e-07 -1.37543883484145e-07 -1.37543912800485e-07;-1.37543883484145e-07 5.75613027339387e-07 -1.37543875208088e-07;-1.37543912800485e-07 -1.37543875208088e-07 5.75613005057695e-07]  x1=[1.0503219260028 9947.75867531084 9948.11570789865;314.159265358979 314.159265358979 314.159265358979;1.19369388127707 -0.103421974588972 -1.67423047603472]  x2=[1.05032249683947 9947.7317058441 9948.08873746365;314.159265358979 314.159265358979 314.159265358979;1.19369263482612 -0.103422348988308 -1.67423085043401]  x3=[0.0142542332217169 534.05471739916 534.073843683364;314.159265358979 314.159265358979 314.159265358979;1.19265369230046 -0.102789665201609 -1.67359816650226]  x4=[0.0142541959883711 536.318767175649 536.337974719093;314.159265358979 314.159265358979 314.159265358979;1.19369077019247 -0.104674895615488 -1.67548339715713]  x5=3.31498451375949e-06  V1=ones(3,3)  V2=ones(3,3)  I1=ones(3,3)  I2=ones(3,3)  nHarmo=1  Measurements=None  Decoupling=off  VsMag0=0  VrMag0=0  VsAngle0=0  VrAngle0=0  IsMag0=0  IrMag0=0  IsAngle0=0  IrAngle0=0
      settings: SourceProductBaseCode=PS
  Line 7 : spsDistributedParametersLineLib/Distributed Parameters Line  Phases=3  Length=1.62  Frequency=50  Resistance=[0.80718830189013 0.0486237908083191 0.0486712220507153;0.0486237908083191 0.807093436079969 0.0486237934466192;0.0486712220507153 0.0486237934466192 0.80718830189013]  Inductance=[0.00279786707424938 0.00133270803418135 0.00132951476746136;0.00133270803418135 0.00279817608385787 0.00133799988507366;0.00132951476746136 0.00133799988507366 0.00279786707424938]  Capacitance=[7.73340098830622e-09 -1.79942827973291e-09 -1.73218055098733e-09;-1.79942827973291e-09 7.66505189233746e-09 -1.83375898618858e-09;-1.73218055098733e-09 -1.83375898618858e-09 7.749673531177e-09]  x1=[54.8229933384025 9848.95271323892 9848.52441391912;314.159265358979 314.159265358979 314.159265358979;1.02286456961992 2.26188396553083 -2.45029819474122]  x2=[54.8233914773796 9848.94148812271 9848.51325335631;314.159265358979 314.159265358979 314.159265358979;1.02286855445759 2.26188048013653 -2.45030169463625]  x3=[0.0478514812800211 24.9236088202226 25.1121990735277;314.159265358979 314.159265358979 314.159265358979;1.01999103409314 2.26027925201648 -2.45190653657412]  x4=[0.047610425347476 24.9616418708861 25.1502335084088;314.159265358979 314.159265358979 314.159265358979;1.02332933308372 2.2615846686665 -2.45059549056523]  x5=7.70442045759223e-06  V1=ones(3,3)  V2=ones(3,3)  I1=ones(3,3)  I2=ones(3,3)  nHarmo=1  Measurements=None  Decoupling=off  VsMag0=0  VrMag0=0  VsAngle0=0  VrAngle0=0  IsMag0=0  IrMag0=0  IsAngle0=0  IrAngle0=0
      settings: SourceProductBaseCode=PS
  Line 70 : spsDistributedParametersLineLib/Distributed Parameters Line  Phases=3  Length=0.50001  Frequency=50  Resistance=[0.646656091154803 0.0486237908083191 0.0486712220507153;0.0486237908083191 0.646561225344642 0.0486237934466192;0.0486712220507153 0.0486237934466192 0.646656091154803]  Inductance=[0.00282448912315926 0.00133270803418135 0.00132951476746136;0.00133270803418135 0.00282479813276775 0.00133799988507366;0.00132951476746136 0.00133799988507366 0.00282448912315926]  Capacitance=[7.89543174552926e-09 -1.85986777702161e-09 -1.7901190036642e-09;-1.85986777702161e-09 7.82540023894543e-09 -1.8957321828871e-09;-1.7901190036642e-09 -1.8957321828871e-09 7.91264394645417e-09]  x1=[130.230707636067 9966.01246212464 9965.41426921905;314.159265358979 314.159265358979 314.159265358979;1.01243318853842 -0.18408725335613 -1.7550486932976]  x2=[130.494546105913 9946.82998998349 9946.30618573429;314.159265358979 314.159265358979 314.159265358979;1.0125571498721 -0.185039367847606 -1.7560010750648]  x3=[0.348475069583015 31.8785270407967 31.6310701858255;314.159265358979 314.159265358979 314.159265358979;0.205750493179934 2.58547305516572 1.02058807177437]  x4=[0.251872240663347 81.1817958226747 81.366212085247;314.159265358979 314.159265358979 314.159265358979;2.63567395015256 -0.327807957744014 -1.89510312007202]  x5=2.3957842710327e-06  V1=ones(3,3)  V2=ones(3,3)  I1=ones(3,3)  I2=ones(3,3)  nHarmo=1  Measurements=None  Decoupling=off  VsMag0=0  VrMag0=0  VsAngle0=0  VrAngle0=0  IsMag0=0  IrMag0=0  IsAngle0=0  IrAngle0=0
      settings: SourceProductBaseCode=PS
